simulink model "model"  (R2014a)
(part 5 of 6)

  bus58 : powerlib/Measurements/Load Flow Bus  LConnTagsString=a  ID=bus58  Vbase=110000  Vref=1  Vangle=0  VLF=1  angleLF=0
      settings: AttributesFormatString=|
      | %<ID>
      | %<Vbase>V
      | %<VLF>pu
      | %<angleLF>deg.
      | %<Name>
  bus580 : powerlib/Measurements/Load Flow Bus  LConnTagsString=a  ID=bus580  Vbase=132000  Vref=1  Vangle=0  VLF=1  angleLF=0
      settings: AttributesFormatString=|
      | %<ID>
      | %<Vbase>V
      | %<VLF>pu
      | %<angleLF>deg.
      | %<Name>
  bus581 : powerlib/Measurements/Load Flow Bus  LConnTagsString=a  ID=bus581  Vbase=132000  Vref=1  Vangle=0  VLF=1  angleLF=0
      settings: AttributesFormatString=|
      | %<ID>
      | %<Vbase>V
      | %<VLF>pu
      | %<angleLF>deg.
      | %<Name>
  bus582 : powerlib/Measurements/Load Flow Bus  LConnTagsString=a  ID=bus582  Vbase=132000  Vref=1  Vangle=0  VLF=1  angleLF=0
      settings: AttributesFormatString=|
      | %<ID>
      | %<Vbase>V
      | %<VLF>pu
      | %<angleLF>deg.
      | %<Name>
  bus583 : powerlib/Measurements/Load Flow Bus  LConnTagsString=a  ID=bus583  Vbase=132000  Vref=1  Vangle=0  VLF=1  angleLF=0
      settings: AttributesFormatString=|
      | %<ID>
      | %<Vbase>V
      | %<VLF>pu
      | %<angleLF>deg.
      | %<Name>
  bus584 : powerlib/Measurements/Load Flow Bus  LConnTagsString=a  ID=bus584  Vbase=132000  Vref=1  Vangle=0  VLF=1  angleLF=0
      settings: AttributesFormatString=|
      | %<ID>
      | %<Vbase>V
      | %<VLF>pu
      | %<angleLF>deg.
      | %<Name>
  bus585 : powerlib/Measurements/Load Flow Bus  LConnTagsString=a  ID=bus585  Vbase=132000  Vref=1  Vangle=0  VLF=1  angleLF=0
      settings: AttributesFormatString=|
      | %<ID>
      | %<Vbase>V
      | %<VLF>pu
      | %<angleLF>deg.
      | %<Name>
  bus586 : powerlib/Measurements/Load Flow Bus  LConnTagsString=a  ID=bus586  Vbase=132000  Vref=1  Vangle=0  VLF=1  angleLF=0
      settings: AttributesFormatString=|
      | %<ID>
      | %<Vbase>V
      | %<VLF>pu
      | %<angleLF>deg.
      | %<Name>
  bus587 : powerlib/Measurements/Load Flow Bus  LConnTagsString=a  ID=bus587  Vbase=132000  Vref=1  Vangle=0  VLF=1  angleLF=0
      settings: AttributesFormatString=|
      | %<ID>
      | %<Vbase>V
      | %<VLF>pu
      | %<angleLF>deg.
      | %<Name>
  bus588 : powerlib/Measurements/Load Flow Bus  LConnTagsString=a  ID=bus588  Vbase=132000  Vref=1  Vangle=0  VLF=1  angleLF=0
      settings: AttributesFormatString=|
      | %<ID>
      | %<Vbase>V
      | %<VLF>pu
      | %<angleLF>deg.
      | %<Name>
  bus589 : powerlib/Measurements/Load Flow Bus  LConnTagsString=a  ID=bus589  Vbase=132000  Vref=1  Vangle=0  VLF=1  angleLF=0
      settings: AttributesFormatString=|
      | %<ID>
      | %<Vbase>V
      | %<VLF>pu
      | %<angleLF>deg.
      | %<Name>
  bus59 : powerlib/Measurements/Load Flow Bus  LConnTagsString=a  ID=bus59  Vbase=110000  Vref=1  Vangle=0  VLF=1  angleLF=0
      settings: AttributesFormatString=|
      | %<ID>
      | %<Vbase>V
      | %<VLF>pu
      | %<angleLF>deg.
      | %<Name>
  bus590 : powerlib/Measurements/Load Flow Bus  LConnTagsString=a  ID=bus590  Vbase=132000  Vref=1  Vangle=0  VLF=1  angleLF=0
      settings: AttributesFormatString=|
      | %<ID>
      | %<Vbase>V
      | %<VLF>pu
      | %<angleLF>deg.
      | %<Name>
  bus591 : powerlib/Measurements/Load Flow Bus  LConnTagsString=a  ID=bus591  Vbase=132000  Vref=1  Vangle=0  VLF=1  angleLF=0
      settings: AttributesFormatString=|
      | %<ID>
      | %<Vbase>V
      | %<VLF>pu
      | %<angleLF>deg.
      | %<Name>
  bus592 : powerlib/Measurements/Load Flow Bus  LConnTagsString=a  ID=bus592  Vbase=132000  Vref=1  Vangle=0  VLF=1  angleLF=0
      settings: AttributesFormatString=|
      | %<ID>
      | %<Vbase>V
      | %<VLF>pu
      | %<angleLF>deg.
      | %<Name>
  bus593 : powerlib/Measurements/Load Flow Bus  LConnTagsString=a  ID=bus593  Vbase=132000  Vref=1  Vangle=0  VLF=1  angleLF=0
      settings: AttributesFormatString=|
      | %<ID>
      | %<Vbase>V
      | %<VLF>pu
      | %<angleLF>deg.
      | %<Name>
  bus594 : powerlib/Measurements/Load Flow Bus  LConnTagsString=a  ID=bus594  Vbase=132000  Vref=1  Vangle=0  VLF=1  angleLF=0
      settings: AttributesFormatString=|
      | %<ID>
      | %<Vbase>V
      | %<VLF>pu
      | %<angleLF>deg.
      | %<Name>
  bus595 : powerlib/Measurements/Load Flow Bus  LConnTagsString=a  ID=bus595  Vbase=132000  Vref=1  Vangle=0  VLF=1  angleLF=0
      settings: AttributesFormatString=|
      | %<ID>
      | %<Vbase>V
      | %<VLF>pu
      | %<angleLF>deg.
      | %<Name>
  bus596 : powerlib/Measurements/Load Flow Bus  LConnTagsString=a  ID=bus596  Vbase=132000  Vref=1  Vangle=0  VLF=1  angleLF=0
      settings: AttributesFormatString=|
      | %<ID>
      | %<Vbase>V
      | %<VLF>pu
      | %<angleLF>deg.
      | %<Name>
  bus597 : powerlib/Measurements/Load Flow Bus  LConnTagsString=a  ID=bus597  Vbase=132000  Vref=1  Vangle=0  VLF=1  angleLF=0
      settings: AttributesFormatString=|
      | %<ID>
      | %<Vbase>V
      | %<VLF>pu
      | %<angleLF>deg.
      | %<Name>
  bus598 : powerlib/Measurements/Load Flow Bus  LConnTagsString=a  ID=bus598  Vbase=132000  Vref=1  Vangle=0  VLF=1  angleLF=0
      settings: AttributesFormatString=|
      | %<ID>
      | %<Vbase>V
      | %<VLF>pu
      | %<angleLF>deg.
      | %<Name>
  bus599 : powerlib/Measurements/Load Flow Bus  LConnTagsString=a  ID=bus599  Vbase=132000  Vref=1  Vangle=0  VLF=1  angleLF=0
      settings: AttributesFormatString=|
      | %<ID>
      | %<Vbase>V
      | %<VLF>pu
      | %<angleLF>deg.
      | %<Name>
  bus6 : powerlib/Measurements/Load Flow Bus  LConnTagsString=a  ID=bus6  Vbase=110000  Vref=1  Vangle=0  VLF=1  angleLF=0
      settings: AttributesFormatString=|
      | %<ID>
      | %<Vbase>V
      | %<VLF>pu
      | %<angleLF>deg.
      | %<Name>
  bus60 : powerlib/Measurements/Load Flow Bus  LConnTagsString=a  ID=bus60  Vbase=110000  Vref=1  Vangle=0  VLF=1  angleLF=0
      settings: AttributesFormatString=|
      | %<ID>
      | %<Vbase>V
      | %<VLF>pu
      | %<angleLF>deg.
      | %<Name>
  bus600 : powerlib/Measurements/Load Flow Bus  LConnTagsString=a  ID=bus600  Vbase=132000  Vref=1  Vangle=0  VLF=1  angleLF=0
      settings: AttributesFormatString=|
      | %<ID>
      | %<Vbase>V
      | %<VLF>pu
      | %<angleLF>deg.
      | %<Name>
  bus601 : powerlib/Measurements/Load Flow Bus  LConnTagsString=a  ID=bus601  Vbase=132000  Vref=1  Vangle=0  VLF=1  angleLF=0
      settings: AttributesFormatString=|
      | %<ID>
      | %<Vbase>V
      | %<VLF>pu
      | %<angleLF>deg.
      | %<Name>
  bus602 : powerlib/Measurements/Load Flow Bus  LConnTagsString=a  ID=bus602  Vbase=132000  Vref=1  Vangle=0  VLF=1  angleLF=0
      settings: AttributesFormatString=|
      | %<ID>
      | %<Vbase>V
      | %<VLF>pu
      | %<angleLF>deg.
      | %<Name>
  bus603 : powerlib/Measurements/Load Flow Bus  LConnTagsString=a  ID=bus603  Vbase=132000  Vref=1  Vangle=0  VLF=1  angleLF=0
      settings: AttributesFormatString=|
      | %<ID>
      | %<Vbase>V
      | %<VLF>pu
      | %<angleLF>deg.
      | %<Name>
  bus604 : powerlib/Measurements/Load Flow Bus  LConnTagsString=a  ID=bus604  Vbase=132000  Vref=1  Vangle=0  VLF=1  angleLF=0
      settings: AttributesFormatString=|
      | %<ID>
      | %<Vbase>V
      | %<VLF>pu
      | %<angleLF>deg.
      | %<Name>
  bus605 : powerlib/Measurements/Load Flow Bus  LConnTagsString=a  ID=bus605  Vbase=132000  Vref=1  Vangle=0  VLF=1  angleLF=0
      settings: AttributesFormatString=|
      | %<ID>
      | %<Vbase>V
      | %<VLF>pu
      | %<angleLF>deg.
      | %<Name>
  bus606 : powerlib/Measurements/Load Flow Bus  LConnTagsString=a  ID=bus606  Vbase=132000  Vref=1  Vangle=0  VLF=1  angleLF=0
      settings: AttributesFormatString=|
      | %<ID>
      | %<Vbase>V
      | %<VLF>pu
      | %<angleLF>deg.
      | %<Name>
  bus607 : powerlib/Measurements/Load Flow Bus  LConnTagsString=a  ID=bus607  Vbase=220000  Vref=1  Vangle=0  VLF=1  angleLF=0
      settings: AttributesFormatString=|
      | %<ID>
      | %<Vbase>V
      | %<VLF>pu
      | %<angleLF>deg.
      | %<Name>
  bus608 : powerlib/Measurements/Load Flow Bus  LConnTagsString=a  ID=bus608  Vbase=220000  Vref=1  Vangle=0  VLF=1  angleLF=0
      settings: AttributesFormatString=|
      | %<ID>
      | %<Vbase>V
      | %<VLF>pu
      | %<angleLF>deg.
      | %<Name>
  bus609 : powerlib/Measurements/Load Flow Bus  LConnTagsString=a  ID=bus609  Vbase=220000  Vref=1  Vangle=0  VLF=1  angleLF=0
      settings: AttributesFormatString=|
      | %<ID>
      | %<Vbase>V
      | %<VLF>pu
      | %<angleLF>deg.
      | %<Name>
  bus61 : powerlib/Measurements/Load Flow Bus  LConnTagsString=a  ID=bus61  Vbase=110000  Vref=1  Vangle=0  VLF=1  angleLF=0
      settings: AttributesFormatString=|
      | %<ID>
      | %<Vbase>V
      | %<VLF>pu
      | %<angleLF>deg.
      | %<Name>
  bus610 : powerlib/Measurements/Load Flow Bus  LConnTagsString=a  ID=bus610  Vbase=220000  Vref=1  Vangle=0  VLF=1  angleLF=0
      settings: AttributesFormatString=|
      | %<ID>
      | %<Vbase>V
      | %<VLF>pu
      | %<angleLF>deg.
      | %<Name>
  bus611 : powerlib/Measurements/Load Flow Bus  LConnTagsString=a  ID=bus611  Vbase=220000  Vref=1  Vangle=0  VLF=1  angleLF=0
      settings: AttributesFormatString=|
      | %<ID>
      | %<Vbase>V
      | %<VLF>pu
      | %<angleLF>deg.
      | %<Name>
  bus612 : powerlib/Measurements/Load Flow Bus  LConnTagsString=a  ID=bus612  Vbase=220000  Vref=1  Vangle=0  VLF=1  angleLF=0
      settings: AttributesFormatString=|
      | %<ID>
      | %<Vbase>V
      | %<VLF>pu
      | %<angleLF>deg.
      | %<Name>
  bus613 : powerlib/Measurements/Load Flow Bus  LConnTagsString=a  ID=bus613  Vbase=220000  Vref=1  Vangle=0  VLF=1  angleLF=0
      settings: AttributesFormatString=|
      | %<ID>
      | %<Vbase>V
      | %<VLF>pu
      | %<angleLF>deg.
      | %<Name>
  bus614 : powerlib/Measurements/Load Flow Bus  LConnTagsString=a  ID=bus614  Vbase=220000  Vref=1  Vangle=0  VLF=1  angleLF=0
      settings: AttributesFormatString=|
      | %<ID>
      | %<Vbase>V
      | %<VLF>pu
      | %<angleLF>deg.
      | %<Name>
  bus615 : powerlib/Measurements/Load Flow Bus  LConnTagsString=a  ID=bus615  Vbase=220000  Vref=1  Vangle=0  VLF=1  angleLF=0
      settings: AttributesFormatString=|
      | %<ID>
      | %<Vbase>V
      | %<VLF>pu
      | %<angleLF>deg.
      | %<Name>
  bus616 : powerlib/Measurements/Load Flow Bus  LConnTagsString=a  ID=bus616  Vbase=220000  Vref=1  Vangle=0  VLF=1  angleLF=0
      settings: AttributesFormatString=|
      | %<ID>
      | %<Vbase>V
      | %<VLF>pu
      | %<angleLF>deg.
      | %<Name>
  bus617 : powerlib/Measurements/Load Flow Bus  LConnTagsString=a  ID=bus617  Vbase=220000  Vref=1  Vangle=0  VLF=1  angleLF=0
      settings: AttributesFormatString=|
      | %<ID>
      | %<Vbase>V
      | %<VLF>pu
      | %<angleLF>deg.
      | %<Name>
  bus618 : powerlib/Measurements/Load Flow Bus  LConnTagsString=a  ID=bus618  Vbase=220000  Vref=1  Vangle=0  VLF=1  angleLF=0
      settings: AttributesFormatString=|
      | %<ID>
      | %<Vbase>V
      | %<VLF>pu
      | %<angleLF>deg.
      | %<Name>
  bus619 : powerlib/Measurements/Load Flow Bus  LConnTagsString=a  ID=bus619  Vbase=220000  Vref=1  Vangle=0  VLF=1  angleLF=0
      settings: AttributesFormatString=|
      | %<ID>
      | %<Vbase>V
      | %<VLF>pu
      | %<angleLF>deg.
      | %<Name>
  bus62 : powerlib/Measurements/Load Flow Bus  LConnTagsString=a  ID=bus62  Vbase=110000  Vref=1  Vangle=0  VLF=1  angleLF=0
      settings: AttributesFormatString=|
      | %<ID>
      | %<Vbase>V
      | %<VLF>pu
      | %<angleLF>deg.
      | %<Name>
  bus620 : powerlib/Measurements/Load Flow Bus  LConnTagsString=a  ID=bus620  Vbase=220000  Vref=1  Vangle=0  VLF=1  angleLF=0
      settings: AttributesFormatString=|
      | %<ID>
      | %<Vbase>V
      | %<VLF>pu
      | %<angleLF>deg.
      | %<Name>
  bus621 : powerlib/Measurements/Load Flow Bus  LConnTagsString=a  ID=bus621  Vbase=220000  Vref=1  Vangle=0  VLF=1  angleLF=0
      settings: AttributesFormatString=|
      | %<ID>
      | %<Vbase>V
      | %<VLF>pu
      | %<angleLF>deg.
      | %<Name>
  bus622 : powerlib/Measurements/Load Flow Bus  LConnTagsString=a  ID=bus622  Vbase=220000  Vref=1  Vangle=0  VLF=1  angleLF=0
      settings: AttributesFormatString=|
      | %<ID>
      | %<Vbase>V
      | %<VLF>pu
      | %<angleLF>deg.
      | %<Name>
  bus623 : powerlib/Measurements/Load Flow Bus  LConnTagsString=a  ID=bus623  Vbase=220000  Vref=1  Vangle=0  VLF=1  angleLF=0
      settings: AttributesFormatString=|
      | %<ID>
      | %<Vbase>V
      | %<VLF>pu
      | %<angleLF>deg.
      | %<Name>
  bus624 : powerlib/Measurements/Load Flow Bus  LConnTagsString=a  ID=bus624  Vbase=220000  Vref=1  Vangle=0  VLF=1  angleLF=0
      settings: AttributesFormatString=|
      | %<ID>
      | %<Vbase>V
      | %<VLF>pu
      | %<angleLF>deg.
      | %<Name>
  bus625 : powerlib/Measurements/Load Flow Bus  LConnTagsString=a  ID=bus625  Vbase=220000  Vref=1  Vangle=0  VLF=1  angleLF=0
      settings: AttributesFormatString=|
      | %<ID>
      | %<Vbase>V
      | %<VLF>pu
      | %<angleLF>deg.
      | %<Name>
  bus626 : powerlib/Measurements/Load Flow Bus  LConnTagsString=a  ID=bus626  Vbase=220000  Vref=1  Vangle=0  VLF=1  angleLF=0
      settings: AttributesFormatString=|
      | %<ID>
      | %<Vbase>V
      | %<VLF>pu
      | %<angleLF>deg.
      | %<Name>
  bus627 : powerlib/Measurements/Load Flow Bus  LConnTagsString=a  ID=bus627  Vbase=220000  Vref=1  Vangle=0  VLF=1  angleLF=0
      settings: AttributesFormatString=|
      | %<ID>
      | %<Vbase>V
      | %<VLF>pu
      | %<angleLF>deg.
      | %<Name>
  bus628 : powerlib/Measurements/Load Flow Bus  LConnTagsString=a  ID=bus628  Vbase=220000  Vref=1  Vangle=0  VLF=1  angleLF=0
      settings: AttributesFormatString=|
      | %<ID>
      | %<Vbase>V
      | %<VLF>pu
      | %<angleLF>deg.
      | %<Name>
  bus629 : powerlib/Measurements/Load Flow Bus  LConnTagsString=a  ID=bus629  Vbase=220000  Vref=1  Vangle=0  VLF=1  angleLF=0
      settings: AttributesFormatString=|
      | %<ID>
      | %<Vbase>V
      | %<VLF>pu
      | %<angleLF>deg.
      | %<Name>
  bus63 : powerlib/Measurements/Load Flow Bus  LConnTagsString=a  ID=bus63  Vbase=110000  Vref=1  Vangle=0  VLF=1  angleLF=0
      settings: AttributesFormatString=|
      | %<ID>
      | %<Vbase>V
      | %<VLF>pu
      | %<angleLF>deg.
      | %<Name>
  bus630 : powerlib/Measurements/Load Flow Bus  LConnTagsString=a  ID=bus630  Vbase=220000  Vref=1  Vangle=0  VLF=1  angleLF=0
      settings: AttributesFormatString=|
      | %<ID>
      | %<Vbase>V
      | %<VLF>pu
      | %<angleLF>deg.
      | %<Name>
  bus631 : powerlib/Measurements/Load Flow Bus  LConnTagsString=a  ID=bus631  Vbase=220000  Vref=1  Vangle=0  VLF=1  angleLF=0
      settings: AttributesFormatString=|
      | %<ID>
      | %<Vbase>V
      | %<VLF>pu
      | %<angleLF>deg.
      | %<Name>
  bus632 : powerlib/Measurements/Load Flow Bus  LConnTagsString=a  ID=bus632  Vbase=220000  Vref=1  Vangle=0  VLF=1  angleLF=0
      settings: AttributesFormatString=|
      | %<ID>
      | %<Vbase>V
      | %<VLF>pu
      | %<angleLF>deg.
      | %<Name>
  bus633 : powerlib/Measurements/Load Flow Bus  LConnTagsString=a  ID=bus633  Vbase=220000  Vref=1  Vangle=0  VLF=1  angleLF=0
      settings: AttributesFormatString=|
      | %<ID>
      | %<Vbase>V
      | %<VLF>pu
      | %<angleLF>deg.
      | %<Name>
  bus634 : powerlib/Measurements/Load Flow Bus  LConnTagsString=a  ID=bus634  Vbase=220000  Vref=1  Vangle=0  VLF=1  angleLF=0
      settings: AttributesFormatString=|
      | %<ID>
      | %<Vbase>V
      | %<VLF>pu
      | %<angleLF>deg.
      | %<Name>
  bus635 : powerlib/Measurements/Load Flow Bus  LConnTagsString=a  ID=bus635  Vbase=220000  Vref=1  Vangle=0  VLF=1  angleLF=0
      settings: AttributesFormatString=|
      | %<ID>
      | %<Vbase>V
      | %<VLF>pu
      | %<angleLF>deg.
      | %<Name>
  bus636 : powerlib/Measurements/Load Flow Bus  LConnTagsString=a  ID=bus636  Vbase=220000  Vref=1  Vangle=0  VLF=1  angleLF=0
      settings: AttributesFormatString=|
      | %<ID>
      | %<Vbase>V
      | %<VLF>pu
      | %<angleLF>deg.
      | %<Name>
  bus637 : powerlib/Measurements/Load Flow Bus  LConnTagsString=a  ID=bus637  Vbase=220000  Vref=1  Vangle=0  VLF=1  angleLF=0
      settings: AttributesFormatString=|
      | %<ID>
      | %<Vbase>V
      | %<VLF>pu
      | %<angleLF>deg.
      | %<Name>
  bus638 : powerlib/Measurements/Load Flow Bus  LConnTagsString=a  ID=bus638  Vbase=220000  Vref=1  Vangle=0  VLF=1  angleLF=0
      settings: AttributesFormatString=|
      | %<ID>
      | %<Vbase>V
      | %<VLF>pu
      | %<angleLF>deg.
      | %<Name>
  bus639 : powerlib/Measurements/Load Flow Bus  LConnTagsString=a  ID=bus639  Vbase=220000  Vref=1  Vangle=0  VLF=1  angleLF=0
      settings: AttributesFormatString=|
      | %<ID>
      | %<Vbase>V
      | %<VLF>pu
      | %<angleLF>deg.
      | %<Name>
  bus64 : powerlib/Measurements/Load Flow Bus  LConnTagsString=a  ID=bus64  Vbase=110000  Vref=1  Vangle=0  VLF=1  angleLF=0
      settings: AttributesFormatString=|
      | %<ID>
      | %<Vbase>V
      | %<VLF>pu
      | %<angleLF>deg.
      | %<Name>
  bus640 : powerlib/Measurements/Load Flow Bus  LConnTagsString=a  ID=bus640  Vbase=220000  Vref=1  Vangle=0  VLF=1  angleLF=0
      settings: AttributesFormatString=|
      | %<ID>
      | %<Vbase>V
      | %<VLF>pu
      | %<angleLF>deg.
      | %<Name>
  bus641 : powerlib/Measurements/Load Flow Bus  LConnTagsString=a  ID=bus641  Vbase=220000  Vref=1  Vangle=0  VLF=1  angleLF=0
      settings: AttributesFormatString=|
      | %<ID>
      | %<Vbase>V
      | %<VLF>pu
      | %<angleLF>deg.
      | %<Name>
  bus642 : powerlib/Measurements/Load Flow Bus  LConnTagsString=a  ID=bus642  Vbase=275000  Vref=1  Vangle=0  VLF=1  angleLF=0
      settings: AttributesFormatString=|
      | %<ID>
      | %<Vbase>V
      | %<VLF>pu
      | %<angleLF>deg.
      | %<Name>
  bus643 : powerlib/Measurements/Load Flow Bus  LConnTagsString=a  ID=bus643  Vbase=275000  Vref=1  Vangle=0  VLF=1  angleLF=0
      settings: AttributesFormatString=|
      | %<ID>
      | %<Vbase>V
      | %<VLF>pu
      | %<angleLF>deg.
      | %<Name>
  bus644 : powerlib/Measurements/Load Flow Bus  LConnTagsString=a  ID=bus644  Vbase=275000  Vref=1  Vangle=0  VLF=1  angleLF=0
      settings: AttributesFormatString=|
      | %<ID>
      | %<Vbase>V
      | %<VLF>pu
      | %<angleLF>deg.
      | %<Name>
  bus645 : powerlib/Measurements/Load Flow Bus  LConnTagsString=a  ID=bus645  Vbase=275000  Vref=1  Vangle=0  VLF=1  angleLF=0
      settings: AttributesFormatString=|
      | %<ID>
      | %<Vbase>V
      | %<VLF>pu
      | %<angleLF>deg.
      | %<Name>
  bus646 : powerlib/Measurements/Load Flow Bus  LConnTagsString=a  ID=bus646  Vbase=275000  Vref=1  Vangle=0  VLF=1  angleLF=0
      settings: AttributesFormatString=|
      | %<ID>
      | %<Vbase>V
      | %<VLF>pu
      | %<angleLF>deg.
      | %<Name>
  bus647 : powerlib/Measurements/Load Flow Bus  LConnTagsString=a  ID=bus647  Vbase=275000  Vref=1  Vangle=0  VLF=1  angleLF=0
      settings: AttributesFormatString=|
      | %<ID>
      | %<Vbase>V
      | %<VLF>pu
      | %<angleLF>deg.
      | %<Name>
  bus648 : powerlib/Measurements/Load Flow Bus  LConnTagsString=a  ID=bus648  Vbase=275000  Vref=1  Vangle=0  VLF=1  angleLF=0
      settings: AttributesFormatString=|
      | %<ID>
      | %<Vbase>V
      | %<VLF>pu
      | %<angleLF>deg.
      | %<Name>
  bus649 : powerlib/Measurements/Load Flow Bus  LConnTagsString=a  ID=bus649  Vbase=275000  Vref=1  Vangle=0  VLF=1  angleLF=0
      settings: AttributesFormatString=|
      | %<ID>
      | %<Vbase>V
      | %<VLF>pu
      | %<angleLF>deg.
      | %<Name>
  bus65 : powerlib/Measurements/Load Flow Bus  LConnTagsString=a  ID=bus65  Vbase=110000  Vref=1  Vangle=0  VLF=1  angleLF=0
      settings: AttributesFormatString=|
      | %<ID>
      | %<Vbase>V
      | %<VLF>pu
      | %<angleLF>deg.
      | %<Name>
  bus650 : powerlib/Measurements/Load Flow Bus  LConnTagsString=a  ID=bus650  Vbase=275000  Vref=1  Vangle=0  VLF=1  angleLF=0
      settings: AttributesFormatString=|
      | %<ID>
      | %<Vbase>V
      | %<VLF>pu
      | %<angleLF>deg.
      | %<Name>
  bus651 : powerlib/Measurements/Load Flow Bus  LConnTagsString=a  ID=bus651  Vbase=275000  Vref=1  Vangle=0  VLF=1  angleLF=0
      settings: AttributesFormatString=|
      | %<ID>
      | %<Vbase>V
      | %<VLF>pu
      | %<angleLF>deg.
      | %<Name>
  bus652 : powerlib/Measurements/Load Flow Bus  LConnTagsString=a  ID=bus652  Vbase=275000  Vref=1  Vangle=0  VLF=1  angleLF=0
      settings: AttributesFormatString=|
      | %<ID>
      | %<Vbase>V
      | %<VLF>pu
      | %<angleLF>deg.
      | %<Name>
  bus653 : powerlib/Measurements/Load Flow Bus  LConnTagsString=a  ID=bus653  Vbase=275000  Vref=1  Vangle=0  VLF=1  angleLF=0
      settings: AttributesFormatString=|
      | %<ID>
      | %<Vbase>V
      | %<VLF>pu
      | %<angleLF>deg.
      | %<Name>
  bus654 : powerlib/Measurements/Load Flow Bus  LConnTagsString=a  ID=bus654  Vbase=275000  Vref=1  Vangle=0  VLF=1  angleLF=0
      settings: AttributesFormatString=|
      | %<ID>
      | %<Vbase>V
      | %<VLF>pu
      | %<angleLF>deg.
      | %<Name>
  bus655 : powerlib/Measurements/Load Flow Bus  LConnTagsString=a  ID=bus655  Vbase=275000  Vref=1  Vangle=0  VLF=1  angleLF=0
      settings: AttributesFormatString=|
      | %<ID>
      | %<Vbase>V
      | %<VLF>pu
      | %<angleLF>deg.
      | %<Name>
  bus656 : powerlib/Measurements/Load Flow Bus  LConnTagsString=a  ID=bus656  Vbase=275000  Vref=1  Vangle=0  VLF=1  angleLF=0
      settings: AttributesFormatString=|
      | %<ID>
      | %<Vbase>V
      | %<VLF>pu
      | %<angleLF>deg.
      | %<Name>
  bus657 : powerlib/Measurements/Load Flow Bus  LConnTagsString=a  ID=bus657  Vbase=275000  Vref=1  Vangle=0  VLF=1  angleLF=0
      settings: AttributesFormatString=|
      | %<ID>
      | %<Vbase>V
      | %<VLF>pu
      | %<angleLF>deg.
      | %<Name>
  bus658 : powerlib/Measurements/Load Flow Bus  LConnTagsString=a  ID=bus658  Vbase=275000  Vref=1  Vangle=0  VLF=1  angleLF=0
      settings: AttributesFormatString=|
      | %<ID>
      | %<Vbase>V
      | %<VLF>pu
      | %<angleLF>deg.
      | %<Name>
  bus659 : powerlib/Measurements/Load Flow Bus  LConnTagsString=a  ID=bus659  Vbase=275000  Vref=1  Vangle=0  VLF=1  angleLF=0
      settings: AttributesFormatString=|
      | %<ID>
      | %<Vbase>V
      | %<VLF>pu
      | %<angleLF>deg.
      | %<Name>
  bus66 : powerlib/Measurements/Load Flow Bus  LConnTagsString=a  ID=bus66  Vbase=110000  Vref=1  Vangle=0  VLF=1  angleLF=0
      settings: AttributesFormatString=|
      | %<ID>
      | %<Vbase>V
      | %<VLF>pu
      | %<angleLF>deg.
      | %<Name>
  bus660 : powerlib/Measurements/Load Flow Bus  LConnTagsString=a  ID=bus660  Vbase=275000  Vref=1  Vangle=0  VLF=1  angleLF=0
      settings: AttributesFormatString=|
      | %<ID>
      | %<Vbase>V
      | %<VLF>pu
      | %<angleLF>deg.
      | %<Name>
  bus661 : powerlib/Measurements/Load Flow Bus  LConnTagsString=a  ID=bus661  Vbase=275000  Vref=1  Vangle=0  VLF=1  angleLF=0
      settings: AttributesFormatString=|
      | %<ID>
      | %<Vbase>V
      | %<VLF>pu
      | %<angleLF>deg.
      | %<Name>
  bus662 : powerlib/Measurements/Load Flow Bus  LConnTagsString=a  ID=bus662  Vbase=275000  Vref=1  Vangle=0  VLF=1  angleLF=0
      settings: AttributesFormatString=|
      | %<ID>
      | %<Vbase>V
      | %<VLF>pu
      | %<angleLF>deg.
      | %<Name>
  bus663 : powerlib/Measurements/Load Flow Bus  LConnTagsString=a  ID=bus663  Vbase=275000  Vref=1  Vangle=0  VLF=1  angleLF=0
      settings: AttributesFormatString=|
      | %<ID>
      | %<Vbase>V
      | %<VLF>pu
      | %<angleLF>deg.
      | %<Name>
  bus664 : powerlib/Measurements/Load Flow Bus  LConnTagsString=a  ID=bus664  Vbase=275000  Vref=1  Vangle=0  VLF=1  angleLF=0
      settings: AttributesFormatString=|
      | %<ID>
      | %<Vbase>V
      | %<VLF>pu
      | %<angleLF>deg.
      | %<Name>
  bus665 : powerlib/Measurements/Load Flow Bus  LConnTagsString=a  ID=bus665  Vbase=275000  Vref=1  Vangle=0  VLF=1  angleLF=0
      settings: AttributesFormatString=|
      | %<ID>
      | %<Vbase>V
      | %<VLF>pu
      | %<angleLF>deg.
      | %<Name>
  bus666 : powerlib/Measurements/Load Flow Bus  LConnTagsString=a  ID=bus666  Vbase=330000  Vref=1  Vangle=0  VLF=1  angleLF=0
      settings: AttributesFormatString=|
      | %<ID>
      | %<Vbase>V
      | %<VLF>pu
      | %<angleLF>deg.
      | %<Name>
  bus667 : powerlib/Measurements/Load Flow Bus  LConnTagsString=a  ID=bus667  Vbase=330000  Vref=1  Vangle=0  VLF=1  angleLF=0
      settings: AttributesFormatString=|
      | %<ID>
      | %<Vbase>V
      | %<VLF>pu
      | %<angleLF>deg.
      | %<Name>
  bus668 : powerlib/Measurements/Load Flow Bus  LConnTagsString=a  ID=bus668  Vbase=330000  Vref=1  Vangle=0  VLF=1  angleLF=0
      settings: AttributesFormatString=|
      | %<ID>
      | %<Vbase>V
      | %<VLF>pu
      | %<angleLF>deg.
      | %<Name>
  bus669 : powerlib/Measurements/Load Flow Bus  LConnTagsString=a  ID=bus669  Vbase=330000  Vref=1  Vangle=0  VLF=1  angleLF=0
      settings: AttributesFormatString=|
      | %<ID>
      | %<Vbase>V
      | %<VLF>pu
      | %<angleLF>deg.
      | %<Name>
  bus67 : powerlib/Measurements/Load Flow Bus  LConnTagsString=a  ID=bus67  Vbase=110000  Vref=1  Vangle=0  VLF=1  angleLF=0
      settings: AttributesFormatString=|
      | %<ID>
      | %<Vbase>V
      | %<VLF>pu
      | %<angleLF>deg.
      | %<Name>
  bus670 : powerlib/Measurements/Load Flow Bus  LConnTagsString=a  ID=bus670  Vbase=330000  Vref=1  Vangle=0  VLF=1  angleLF=0
      settings: AttributesFormatString=|
      | %<ID>
      | %<Vbase>V
      | %<VLF>pu
      | %<angleLF>deg.
      | %<Name>
  bus671 : powerlib/Measurements/Load Flow Bus  LConnTagsString=a  ID=bus671  Vbase=330000  Vref=1  Vangle=0  VLF=1  angleLF=0
      settings: AttributesFormatString=|
      | %<ID>
      | %<Vbase>V
      | %<VLF>pu
      | %<angleLF>deg.
      | %<Name>
  bus672 : powerlib/Measurements/Load Flow Bus  LConnTagsString=a  ID=bus672  Vbase=330000  Vref=1  Vangle=0  VLF=1  angleLF=0
      settings: AttributesFormatString=|
      | %<ID>
      | %<Vbase>V
      | %<VLF>pu
      | %<angleLF>deg.
      | %<Name>
  bus673 : powerlib/Measurements/Load Flow Bus  LConnTagsString=a  ID=bus673  Vbase=330000  Vref=1  Vangle=0  VLF=1  angleLF=0
      settings: AttributesFormatString=|
      | %<ID>
      | %<Vbase>V
      | %<VLF>pu
      | %<angleLF>deg.
      | %<Name>
  bus674 : powerlib/Measurements/Load Flow Bus  LConnTagsString=a  ID=bus674  Vbase=330000  Vref=1  Vangle=0  VLF=1  angleLF=0
      settings: AttributesFormatString=|
      | %<ID>
      | %<Vbase>V
      | %<VLF>pu
      | %<angleLF>deg.
      | %<Name>
  bus675 : powerlib/Measurements/Load Flow Bus  LConnTagsString=a  ID=bus675  Vbase=330000  Vref=1  Vangle=0  VLF=1  angleLF=0
      settings: AttributesFormatString=|
      | %<ID>
      | %<Vbase>V
      | %<VLF>pu
      | %<angleLF>deg.
      | %<Name>
  bus676 : powerlib/Measurements/Load Flow Bus  LConnTagsString=a  ID=bus676  Vbase=330000  Vref=1  Vangle=0  VLF=1  angleLF=0
      settings: AttributesFormatString=|
      | %<ID>
      | %<Vbase>V
      | %<VLF>pu
      | %<angleLF>deg.
      | %<Name>
  bus677 : powerlib/Measurements/Load Flow Bus  LConnTagsString=a  ID=bus677  Vbase=330000  Vref=1  Vangle=0  VLF=1  angleLF=0
      settings: AttributesFormatString=|
      | %<ID>
      | %<Vbase>V
      | %<VLF>pu
      | %<angleLF>deg.
      | %<Name>
  bus678 : powerlib/Measurements/Load Flow Bus  LConnTagsString=a  ID=bus678  Vbase=330000  Vref=1  Vangle=0  VLF=1  angleLF=0
      settings: AttributesFormatString=|
      | %<ID>
      | %<Vbase>V
      | %<VLF>pu
      | %<angleLF>deg.
      | %<Name>
  bus679 : powerlib/Measurements/Load Flow Bus  LConnTagsString=a  ID=bus679  Vbase=330000  Vref=1  Vangle=0  VLF=1  angleLF=0
      settings: AttributesFormatString=|
      | %<ID>
      | %<Vbase>V
      | %<VLF>pu
      | %<angleLF>deg.
      | %<Name>
  bus68 : powerlib/Measurements/Load Flow Bus  LConnTagsString=a  ID=bus68  Vbase=132000  Vref=1  Vangle=0  VLF=1  angleLF=0
      settings: AttributesFormatString=|
      | %<ID>
      | %<Vbase>V
      | %<VLF>pu
      | %<angleLF>deg.
      | %<Name>
  bus680 : powerlib/Measurements/Load Flow Bus  LConnTagsString=a  ID=bus680  Vbase=330000  Vref=1  Vangle=0  VLF=1  angleLF=0
      settings: AttributesFormatString=|
      | %<ID>
      | %<Vbase>V
      | %<VLF>pu
      | %<angleLF>deg.
      | %<Name>
  bus681 : powerlib/Measurements/Load Flow Bus  LConnTagsString=a  ID=bus681  Vbase=330000  Vref=1  Vangle=0  VLF=1  angleLF=0
      settings: AttributesFormatString=|
      | %<ID>
      | %<Vbase>V
      | %<VLF>pu
      | %<angleLF>deg.
      | %<Name>
  bus682 : powerlib/Measurements/Load Flow Bus  LConnTagsString=a  ID=bus682  Vbase=330000  Vref=1  Vangle=0  VLF=1  angleLF=0
      settings: AttributesFormatString=|
      | %<ID>
      | %<Vbase>V
      | %<VLF>pu
      | %<angleLF>deg.
      | %<Name>
  bus683 : powerlib/Measurements/Load Flow Bus  LConnTagsString=a  ID=bus683  Vbase=330000  Vref=1  Vangle=0  VLF=1  angleLF=0
      settings: AttributesFormatString=|
      | %<ID>
      | %<Vbase>V
      | %<VLF>pu
      | %<angleLF>deg.
      | %<Name>
  bus684 : powerlib/Measurements/Load Flow Bus  LConnTagsString=a  ID=bus684  Vbase=330000  Vref=1  Vangle=0  VLF=1  angleLF=0
      settings: AttributesFormatString=|
      | %<ID>
      | %<Vbase>V
      | %<VLF>pu
      | %<angleLF>deg.
      | %<Name>
  bus685 : powerlib/Measurements/Load Flow Bus  LConnTagsString=a  ID=bus685  Vbase=330000  Vref=1  Vangle=0  VLF=1  angleLF=0
      settings: AttributesFormatString=|
      | %<ID>
      | %<Vbase>V
      | %<VLF>pu
      | %<angleLF>deg.
      | %<Name>
  bus686 : powerlib/Measurements/Load Flow Bus  LConnTagsString=a  ID=bus686  Vbase=330000  Vref=1  Vangle=0  VLF=1  angleLF=0
      settings: AttributesFormatString=|
      | %<ID>
      | %<Vbase>V
      | %<VLF>pu
      | %<angleLF>deg.
      | %<Name>
  bus687 : powerlib/Measurements/Load Flow Bus  LConnTagsString=a  ID=bus687  Vbase=330000  Vref=1  Vangle=0  VLF=1  angleLF=0
      settings: AttributesFormatString=|
      | %<ID>
      | %<Vbase>V
      | %<VLF>pu
      | %<angleLF>deg.
      | %<Name>
  bus688 : powerlib/Measurements/Load Flow Bus  LConnTagsString=a  ID=bus688  Vbase=330000  Vref=1  Vangle=0  VLF=1  angleLF=0
      settings: AttributesFormatString=|
      | %<ID>
      | %<Vbase>V
      | %<VLF>pu
      | %<angleLF>deg.
      | %<Name>
  bus689 : powerlib/Measurements/Load Flow Bus  LConnTagsString=a  ID=bus689  Vbase=500000  Vref=1  Vangle=0  VLF=1  angleLF=0
      settings: AttributesFormatString=|
      | %<ID>
      | %<Vbase>V
      | %<VLF>pu
      | %<angleLF>deg.
      | %<Name>
  bus69 : powerlib/Measurements/Load Flow Bus  LConnTagsString=a  ID=bus69  Vbase=132000  Vref=1  Vangle=0  VLF=1  angleLF=0
      settings: AttributesFormatString=|
      | %<ID>
      | %<Vbase>V
      | %<VLF>pu
      | %<angleLF>deg.
      | %<Name>
  bus690 : powerlib/Measurements/Load Flow Bus  LConnTagsString=a  ID=bus690  Vbase=500000  Vref=1  Vangle=0  VLF=1  angleLF=0
      settings: AttributesFormatString=|
      | %<ID>
      | %<Vbase>V
      | %<VLF>pu
      | %<angleLF>deg.
      | %<Name>
  bus691 : powerlib/Measurements/Load Flow Bus  LConnTagsString=a  ID=bus691  Vbase=500000  Vref=1  Vangle=0  VLF=1  angleLF=0
      settings: AttributesFormatString=|
      | %<ID>
      | %<Vbase>V
      | %<VLF>pu
      | %<angleLF>deg.
      | %<Name>
  bus692 : powerlib/Measurements/Load Flow Bus  LConnTagsString=a  ID=bus692  Vbase=500000  Vref=1  Vangle=0  VLF=1  angleLF=0
      settings: AttributesFormatString=|
      | %<ID>
      | %<Vbase>V
      | %<VLF>pu
      | %<angleLF>deg.
      | %<Name>
  bus693 : powerlib/Measurements/Load Flow Bus  LConnTagsString=a  ID=bus693  Vbase=500000  Vref=1  Vangle=0  VLF=1  angleLF=0
      settings: AttributesFormatString=|
      | %<ID>
      | %<Vbase>V
      | %<VLF>pu
      | %<angleLF>deg.
      | %<Name>
  bus694 : powerlib/Measurements/Load Flow Bus  LConnTagsString=a  ID=bus694  Vbase=500000  Vref=1  Vangle=0  VLF=1  angleLF=0
      settings: AttributesFormatString=|
      | %<ID>
      | %<Vbase>V
      | %<VLF>pu
      | %<angleLF>deg.
      | %<Name>
  bus7 : powerlib/Measurements/Load Flow Bus  LConnTagsString=a  ID=bus7  Vbase=110000  Vref=1  Vangle=0  VLF=1  angleLF=0
      settings: AttributesFormatString=|
      | %<ID>
      | %<Vbase>V
      | %<VLF>pu
      | %<angleLF>deg.
      | %<Name>
  bus70 : powerlib/Measurements/Load Flow Bus  LConnTagsString=a  ID=bus70  Vbase=132000  Vref=1  Vangle=0  VLF=1  angleLF=0
      settings: AttributesFormatString=|
      | %<ID>
      | %<Vbase>V
      | %<VLF>pu
      | %<angleLF>deg.
      | %<Name>
  bus71 : powerlib/Measurements/Load Flow Bus  LConnTagsString=a  ID=bus71  Vbase=132000  Vref=1  Vangle=0  VLF=1  angleLF=0
      settings: AttributesFormatString=|
      | %<ID>
      | %<Vbase>V
      | %<VLF>pu
      | %<angleLF>deg.
      | %<Name>
  bus72 : powerlib/Measurements/Load Flow Bus  LConnTagsString=a  ID=bus72  Vbase=132000  Vref=1  Vangle=0  VLF=1  angleLF=0
      settings: AttributesFormatString=|
      | %<ID>
      | %<Vbase>V
      | %<VLF>pu
      | %<angleLF>deg.
      | %<Name>
  bus73 : powerlib/Measurements/Load Flow Bus  LConnTagsString=a  ID=bus73  Vbase=132000  Vref=1  Vangle=0  VLF=1  angleLF=0
      settings: AttributesFormatString=|
      | %<ID>
      | %<Vbase>V
      | %<VLF>pu
      | %<angleLF>deg.
      | %<Name>
  bus74 : powerlib/Measurements/Load Flow Bus  LConnTagsString=a  ID=bus74  Vbase=132000  Vref=1  Vangle=0  VLF=1  angleLF=0
      settings: AttributesFormatString=|
      | %<ID>
      | %<Vbase>V
      | %<VLF>pu
      | %<angleLF>deg.
      | %<Name>
  bus75 : powerlib/Measurements/Load Flow Bus  LConnTagsString=a  ID=bus75  Vbase=132000  Vref=1  Vangle=0  VLF=1  angleLF=0
      settings: AttributesFormatString=|
      | %<ID>
      | %<Vbase>V
      | %<VLF>pu
      | %<angleLF>deg.
      | %<Name>
  bus76 : powerlib/Measurements/Load Flow Bus  LConnTagsString=a  ID=bus76  Vbase=132000  Vref=1  Vangle=0  VLF=1  angleLF=0
      settings: AttributesFormatString=|
      | %<ID>
      | %<Vbase>V
      | %<VLF>pu
      | %<angleLF>deg.
      | %<Name>
  bus77 : powerlib/Measurements/Load Flow Bus  LConnTagsString=a  ID=bus77  Vbase=132000  Vref=1  Vangle=0  VLF=1  angleLF=0
      settings: AttributesFormatString=|
      | %<ID>
      | %<Vbase>V
      | %<VLF>pu
      | %<angleLF>deg.
      | %<Name>
  bus78 : powerlib/Measurements/Load Flow Bus  LConnTagsString=a  ID=bus78  Vbase=132000  Vref=1  Vangle=0  VLF=1  angleLF=0
      settings: AttributesFormatString=|
      | %<ID>
      | %<Vbase>V
      | %<VLF>pu
      | %<angleLF>deg.
      | %<Name>
  bus79 : powerlib/Measurements/Load Flow Bus  LConnTagsString=a  ID=bus79  Vbase=132000  Vref=1  Vangle=0  VLF=1  angleLF=0
      settings: AttributesFormatString=|
      | %<ID>
      | %<Vbase>V
      | %<VLF>pu
      | %<angleLF>deg.
      | %<Name>
  bus8 : powerlib/Measurements/Load Flow Bus  LConnTagsString=a  ID=bus8  Vbase=110000  Vref=1  Vangle=0  VLF=1  angleLF=0
      settings: AttributesFormatString=|
      | %<ID>
      | %<Vbase>V
      | %<VLF>pu
      | %<angleLF>deg.
      | %<Name>
  bus80 : powerlib/Measurements/Load Flow Bus  LConnTagsString=a  ID=bus80  Vbase=132000  Vref=1  Vangle=0  VLF=1  angleLF=0
      settings: AttributesFormatString=|
      | %<ID>
      | %<Vbase>V
      | %<VLF>pu
      | %<angleLF>deg.
      | %<Name>
  bus81 : powerlib/Measurements/Load Flow Bus  LConnTagsString=a  ID=bus81  Vbase=132000  Vref=1  Vangle=0  VLF=1  angleLF=0
      settings: AttributesFormatString=|
      | %<ID>
      | %<Vbase>V
      | %<VLF>pu
      | %<angleLF>deg.
      | %<Name>
  bus82 : powerlib/Measurements/Load Flow Bus  LConnTagsString=a  ID=bus82  Vbase=132000  Vref=1  Vangle=0  VLF=1  angleLF=0
      settings: AttributesFormatString=|
      | %<ID>
      | %<Vbase>V
      | %<VLF>pu
      | %<angleLF>deg.
      | %<Name>
  bus83 : powerlib/Measurements/Load Flow Bus  LConnTagsString=a  ID=bus83  Vbase=132000  Vref=1  Vangle=0  VLF=1  angleLF=0
      settings: AttributesFormatString=|
      | %<ID>
      | %<Vbase>V
      | %<VLF>pu
      | %<angleLF>deg.
      | %<Name>
  bus84 : powerlib/Measurements/Load Flow Bus  LConnTagsString=a  ID=bus84  Vbase=132000  Vref=1  Vangle=0  VLF=1  angleLF=0
      settings: AttributesFormatString=|
      | %<ID>
      | %<Vbase>V
      | %<VLF>pu
      | %<angleLF>deg.
      | %<Name>
  bus85 : powerlib/Measurements/Load Flow Bus  LConnTagsString=a  ID=bus85  Vbase=132000  Vref=1  Vangle=0  VLF=1  angleLF=0
      settings: AttributesFormatString=|
      | %<ID>
      | %<Vbase>V
      | %<VLF>pu
      | %<angleLF>deg.
      | %<Name>
  bus86 : powerlib/Measurements/Load Flow Bus  LConnTagsString=a  ID=bus86  Vbase=132000  Vref=1  Vangle=0  VLF=1  angleLF=0
      settings: AttributesFormatString=|
      | %<ID>
      | %<Vbase>V
      | %<VLF>pu
      | %<angleLF>deg.
      | %<Name>
  bus87 : powerlib/Measurements/Load Flow Bus  LConnTagsString=a  ID=bus87  Vbase=132000  Vref=1  Vangle=0  VLF=1  angleLF=0
      settings: AttributesFormatString=|
      | %<ID>
      | %<Vbase>V
      | %<VLF>pu
      | %<angleLF>deg.
      | %<Name>
  bus88 : powerlib/Measurements/Load Flow Bus  LConnTagsString=a  ID=bus88  Vbase=132000  Vref=1  Vangle=0  VLF=1  angleLF=0
      settings: AttributesFormatString=|
      | %<ID>
      | %<Vbase>V
      | %<VLF>pu
      | %<angleLF>deg.
      | %<Name>
  bus89 : powerlib/Measurements/Load Flow Bus  LConnTagsString=a  ID=bus89  Vbase=132000  Vref=1  Vangle=0  VLF=1  angleLF=0
      settings: AttributesFormatString=|
      | %<ID>
      | %<Vbase>V
      | %<VLF>pu
      | %<angleLF>deg.
      | %<Name>
  bus9 : powerlib/Measurements/Load Flow Bus  LConnTagsString=a  ID=bus9  Vbase=110000  Vref=1  Vangle=0  VLF=1  angleLF=0
      settings: AttributesFormatString=|
      | %<ID>
      | %<Vbase>V
      | %<VLF>pu
      | %<angleLF>deg.
      | %<Name>
  bus90 : powerlib/Measurements/Load Flow Bus  LConnTagsString=a  ID=bus90  Vbase=132000  Vref=1  Vangle=0  VLF=1  angleLF=0
      settings: AttributesFormatString=|
      | %<ID>
      | %<Vbase>V
      | %<VLF>pu
      | %<angleLF>deg.
      | %<Name>
  bus91 : powerlib/Measurements/Load Flow Bus  LConnTagsString=a  ID=bus91  Vbase=132000  Vref=1  Vangle=0  VLF=1  angleLF=0
      settings: AttributesFormatString=|
      | %<ID>
      | %<Vbase>V
      | %<VLF>pu
      | %<angleLF>deg.
      | %<Name>
  bus92 : powerlib/Measurements/Load Flow Bus  LConnTagsString=a  ID=bus92  Vbase=132000  Vref=1  Vangle=0  VLF=1  angleLF=0
      settings: AttributesFormatString=|
      | %<ID>
      | %<Vbase>V
      | %<VLF>pu
      | %<angleLF>deg.
      | %<Name>
  bus93 : powerlib/Measurements/Load Flow Bus  LConnTagsString=a  ID=bus93  Vbase=132000  Vref=1  Vangle=0  VLF=1  angleLF=0
      settings: AttributesFormatString=|
      | %<ID>
      | %<Vbase>V
      | %<VLF>pu
      | %<angleLF>deg.
      | %<Name>
  bus94 : powerlib/Measurements/Load Flow Bus  LConnTagsString=a  ID=bus94  Vbase=132000  Vref=1  Vangle=0  VLF=1  angleLF=0
      settings: AttributesFormatString=|
      | %<ID>
      | %<Vbase>V
      | %<VLF>pu
      | %<angleLF>deg.
      | %<Name>
  bus95 : powerlib/Measurements/Load Flow Bus  LConnTagsString=a  ID=bus95  Vbase=132000  Vref=1  Vangle=0  VLF=1  angleLF=0
      settings: AttributesFormatString=|
      | %<ID>
      | %<Vbase>V
      | %<VLF>pu
      | %<angleLF>deg.
      | %<Name>
  bus96 : powerlib/Measurements/Load Flow Bus  LConnTagsString=a  ID=bus96  Vbase=132000  Vref=1  Vangle=0  VLF=1  angleLF=0
      settings: AttributesFormatString=|
      | %<ID>
      | %<Vbase>V
      | %<VLF>pu
      | %<angleLF>deg.
      | %<Name>
  bus97 : powerlib/Measurements/Load Flow Bus  LConnTagsString=a  ID=bus97  Vbase=132000  Vref=1  Vangle=0  VLF=1  angleLF=0
      settings: AttributesFormatString=|
      | %<ID>
      | %<Vbase>V
      | %<VLF>pu
      | %<angleLF>deg.
      | %<Name>
  bus98 : powerlib/Measurements/Load Flow Bus  LConnTagsString=a  ID=bus98  Vbase=132000  Vref=1  Vangle=0  VLF=1  angleLF=0
      settings: AttributesFormatString=|
      | %<ID>
      | %<Vbase>V
      | %<VLF>pu
      | %<angleLF>deg.
      | %<Name>
  bus99 : powerlib/Measurements/Load Flow Bus  LConnTagsString=a  ID=bus99  Vbase=132000  Vref=1  Vangle=0  VLF=1  angleLF=0
      settings: AttributesFormatString=|
      | %<ID>
      | %<Vbase>V
      | %<VLF>pu
      | %<angleLF>deg.
      | %<Name>
  powergui : powerlib/powergui  Priority=1  SimulationMode=Continuous  SolverType=Tustin  SampleTime=50e-6  frequency=60  SPID=off  DisableSnubberDevices=off  DisableRonSwitches=off  DisableVfSwitches=off  SwTol=0  Interpol=off  DisplayEquations=off  Ts=0  methode=off  frequencyindice=60  Pbase=100e6  ErrMax=1e-4  Iterations=50  UnitsV=kV  UnitsW=MW  FunctionMessages=off  echomessages=off  HookPort=off  EnableUseOfTLC=off  x0status=blocks  RestoreLinks=warning  ResistiveCurrentMeasurement=off  Frange=[0:2:500]  Ylog=off  Xlog=on  ShowGrid=off  save=off  variable=ZData  structure=0  ZoomFFT=off  StartTime=0.0  cycles=1  DisplayStyle=1  fundamental=60  FreqAxis=off  MaxFrequency=1000  frequencyindicesteady=1  RmsSteady=1  display=off
  connections:
  T_305092097__/LConn1 -- _CN_305092097_110000_CN_305092094_110000/LConn1
  T_305092097__/LConn2 -- _CN_305092097_110000_CN_305092094_110000/LConn2
  _CN_305092097_110000_CN_305092094_110000/LConn3 -- T_305092097__/LConn3 -- bus1/LConn1
  T_305092094__/LConn1 -- _CN_305092097_110000_CN_305092094_110000/RConn1
  T_305092094__/LConn2 -- _CN_305092097_110000_CN_305092094_110000/RConn2
  _CN_305092097_110000_CN_305092094_110000/RConn3 -- T_305092094__/LConn3 -- bus2/LConn1
  _CN_88187651_110000_CN_61649117_110000/LConn1 -- T_88187651__Hadspen_Substation/RConn1 -- _CN_88187651_110000_CN_174441055_110000/LConn1 -- L_88187651/LConn1
  _CN_88187651_110000_CN_61649117_110000/LConn2 -- T_88187651__Hadspen_Substation/RConn2 -- _CN_88187651_110000_CN_174441055_110000/LConn2 -- L_88187651/LConn2
  _CN_88187651_110000_CN_61649117_110000/LConn3 -- T_88187651__Hadspen_Substation/RConn3 -- _CN_88187651_110000_CN_174441055_110000/LConn3 -- L_88187651/LConn3 -- bus3/LConn1
  G_61649117_Trevallyn_Power_Station/RConn1 -- _CN_88187651_110000_CN_61649117_110000/RConn1
  G_61649117_Trevallyn_Power_Station/RConn2 -- _CN_88187651_110000_CN_61649117_110000/RConn2
  _CN_88187651_110000_CN_61649117_110000/RConn3 -- G_61649117_Trevallyn_Power_Station/RConn3 -- bus4/LConn1
  _CN_88187651_110000_CN_174441055_110000/RConn1 -- T_174441055__/RConn1 -- L_174441055/LConn1
  _CN_88187651_110000_CN_174441055_110000/RConn2 -- T_174441055__/RConn2 -- L_174441055/LConn2
  _CN_88187651_110000_CN_174441055_110000/RConn3 -- T_174441055__/RConn3 -- L_174441055/LConn3 -- bus5/LConn1
  _CN_303420374_110000_CN_46146107_110000/LConn1 -- T_303420374__Richlands_Substation/LConn1 -- _CN_303420374_110000_CN_19388439_110000/LConn1 -- _CN_303420374_110000_CN_303417152_110000/LConn1
  _CN_303420374_110000_CN_46146107_110000/LConn2 -- T_303420374__Richlands_Substation/LConn2 -- _CN_303420374_110000_CN_19388439_110000/LConn2 -- _CN_303420374_110000_CN_303417152_110000/LConn2
  _CN_303420374_110000_CN_46146107_110000/LConn3 -- T_303420374__Richlands_Substation/LConn3 -- _CN_303420374_110000_CN_19388439_110000/LConn3 -- _CN_303420374_110000_CN_303417152_110000/LConn3 -- bus6/LConn1
  _CN_303420374_110000_CN_46146107_110000/RConn1 -- T_46146107__Algester_Substation/LConn1 -- _CN_26161587_110000_CN_46146107_110000/LConn1
  _CN_303420374_110000_CN_46146107_110000/RConn2 -- T_46146107__Algester_Substation/LConn2 -- _CN_26161587_110000_CN_46146107_110000/LConn2
  _CN_303420374_110000_CN_46146107_110000/RConn3 -- T_46146107__Algester_Substation/LConn3 -- _CN_26161587_110000_CN_46146107_110000/LConn3 -- bus7/LConn1
  _CN_303420374_110000_CN_19388439_110000/RConn1 -- T_19388439__West_Darra_Substation/LConn1 -- _CN_19388439_110000_CN_173223683_110000/LConn1 -- _CN_19388439_110000_CN_19386719_110000/LConn1 -- _CN_19388439_110000_CN_46305863_110000/LConn1
  _CN_303420374_110000_CN_19388439_110000/RConn2 -- T_19388439__West_Darra_Substation/LConn2 -- _CN_19388439_110000_CN_173223683_110000/LConn2 -- _CN_19388439_110000_CN_19386719_110000/LConn2 -- _CN_19388439_110000_CN_46305863_110000/LConn2
  _CN_303420374_110000_CN_19388439_110000/RConn3 -- T_19388439__West_Darra_Substation/LConn3 -- _CN_19388439_110000_CN_173223683_110000/LConn3 -- _CN_19388439_110000_CN_19386719_110000/LConn3 -- bus8/LConn1 -- _CN_19388439_110000_CN_46305863_110000/LConn3
  T_303417152__Sumner_Substation/LConn1 -- _CN_303420374_110000_CN_303417152_110000/RConn1
  T_303417152__Sumner_Substation/LConn2 -- _CN_303420374_110000_CN_303417152_110000/RConn2
  _CN_303420374_110000_CN_303417152_110000/RConn3 -- T_303417152__Sumner_Substation/LConn3 -- bus9/LConn1
  T_162321863__/LConn1 -- _CN_162321863_110000_CN_19380255_110000/LConn1
  T_162321863__/LConn2 -- _CN_162321863_110000_CN_19380255_110000/LConn2
  _CN_162321863_110000_CN_19380255_110000/LConn3 -- T_162321863__/LConn3 -- bus10/LConn1
  _CN_162321863_110000_CN_19380255_110000/RConn1 -- G_19380255_Swanbank_Power_Station/RConn1 -- _CN_173223683_110000_CN_19380255_110000/LConn1 -- _CN_170832455_275000_CN_19380255_110000/LConn1
  _CN_162321863_110000_CN_19380255_110000/RConn2 -- G_19380255_Swanbank_Power_Station/RConn2 -- _CN_173223683_110000_CN_19380255_110000/LConn2 -- _CN_170832455_275000_CN_19380255_110000/LConn2
  _CN_162321863_110000_CN_19380255_110000/RConn3 -- G_19380255_Swanbank_Power_Station/RConn3 -- _CN_173223683_110000_CN_19380255_110000/LConn3 -- _CN_170832455_275000_CN_19380255_110000/LConn3 -- bus11/LConn1
  T_372546567__/LConn1 -- _CN_372546567_110000_CN_23171307_110000/LConn1
  T_372546567__/LConn2 -- _CN_372546567_110000_CN_23171307_110000/LConn2
  _CN_372546567_110000_CN_23171307_110000/LConn3 -- T_372546567__/LConn3 -- bus12/LConn1
  T_23171307__/LConn1 -- _CN_372546567_110000_CN_23171307_110000/RConn1
  T_23171307__/LConn2 -- _CN_372546567_110000_CN_23171307_110000/RConn2
  _CN_372546567_110000_CN_23171307_110000/RConn3 -- T_23171307__/LConn3 -- bus13/LConn1
  T_233929226__/LConn1 -- _CN_233929226_110000_CN_435794582_110000/LConn1
  T_233929226__/LConn2 -- _CN_233929226_110000_CN_435794582_110000/LConn2
  _CN_233929226_110000_CN_435794582_110000/LConn3 -- T_233929226__/LConn3 -- bus14/LConn1
  _CN_233929226_110000_CN_435794582_110000/RConn1 -- T_435794582__Tungatinah_Switchyard/LConn1 -- _CN_435794582_110000_CN_176275951_110000/LConn1
  _CN_233929226_110000_CN_435794582_110000/RConn2 -- T_435794582__Tungatinah_Switchyard/LConn2 -- _CN_435794582_110000_CN_176275951_110000/LConn2
  _CN_233929226_110000_CN_435794582_110000/RConn3 -- T_435794582__Tungatinah_Switchyard/LConn3 -- _CN_435794582_110000_CN_176275951_110000/LConn3 -- bus15/LConn1
  _CN_23298443_110000_CN_23239876_110000/LConn1 -- T_23298443__/RConn1 -- _CN_23298443_110000_CN_175926350_110000/LConn1 -- _CN_23298443_110000_CN_233927398_110000/LConn1 -- _CN_23298443_110000_CN_233927458_110000/LConn1 -- L_23298443/LConn1
  _CN_23298443_110000_CN_23239876_110000/LConn2 -- T_23298443__/RConn2 -- _CN_23298443_110000_CN_175926350_110000/LConn2 -- _CN_23298443_110000_CN_233927398_110000/LConn2 -- _CN_23298443_110000_CN_233927458_110000/LConn2 -- L_23298443/LConn2
  _CN_23298443_110000_CN_23239876_110000/LConn3 -- T_23298443__/RConn3 -- _CN_23298443_110000_CN_175926350_110000/LConn3 -- _CN_23298443_110000_CN_233927398_110000/LConn3 -- _CN_23298443_110000_CN_233927458_110000/LConn3 -- L_23298443/LConn3 -- bus16/LConn1
  T_23239876__/LConn1 -- _CN_23298443_110000_CN_23239876_110000/RConn1
  T_23239876__/LConn2 -- _CN_23298443_110000_CN_23239876_110000/RConn2
  _CN_23298443_110000_CN_23239876_110000/RConn3 -- T_23239876__/LConn3 -- bus17/LConn1
  _CN_23298443_110000_CN_175926350_110000/RConn1 -- T_175926350__/LConn1 -- _CN_175926345_110000_CN_175926350_110000/LConn1
  _CN_23298443_110000_CN_175926350_110000/RConn2 -- T_175926350__/LConn2 -- _CN_175926345_110000_CN_175926350_110000/LConn2
  _CN_23298443_110000_CN_175926350_110000/RConn3 -- T_175926350__/LConn3 -- _CN_175926345_110000_CN_175926350_110000/LConn3 -- bus18/LConn1
  T_233927398__/LConn1 -- _CN_23298443_110000_CN_233927398_110000/RConn1
  T_233927398__/LConn2 -- _CN_23298443_110000_CN_233927398_110000/RConn2
  _CN_23298443_110000_CN_233927398_110000/RConn3 -- T_233927398__/LConn3 -- bus19/LConn1
  T_233927458__/LConn1 -- _CN_23298443_110000_CN_233927458_110000/RConn1
  T_233927458__/LConn2 -- _CN_23298443_110000_CN_233927458_110000/RConn2
  _CN_23298443_110000_CN_233927458_110000/RConn3 -- T_233927458__/LConn3 -- bus20/LConn1
  T_374644110__/LConn1 -- _CN_374644110_110000_CN_46056595_110000/LConn1
  T_374644110__/LConn2 -- _CN_374644110_110000_CN_46056595_110000/LConn2
  _CN_374644110_110000_CN_46056595_110000/LConn3 -- T_374644110__/LConn3 -- bus21/LConn1
  T_46056595__/LConn1 -- _CN_374644110_110000_CN_46056595_110000/RConn1
  T_46056595__/LConn2 -- _CN_374644110_110000_CN_46056595_110000/RConn2
  _CN_374644110_110000_CN_46056595_110000/RConn3 -- T_46056595__/LConn3 -- bus22/LConn1
  _CN_19384720_110000_CN_171582113_110000/LConn1 -- T_19384720__South_Pine_Substation/RConn1 -- L_19384720/LConn1
  _CN_19384720_110000_CN_171582113_110000/LConn2 -- T_19384720__South_Pine_Substation/RConn2 -- L_19384720/LConn2
  _CN_19384720_110000_CN_171582113_110000/LConn3 -- T_19384720__South_Pine_Substation/RConn3 -- L_19384720/LConn3 -- bus23/LConn1
  T_171582113__/LConn1 -- _CN_19384720_110000_CN_171582113_110000/RConn1
  T_171582113__/LConn2 -- _CN_19384720_110000_CN_171582113_110000/RConn2
  _CN_19384720_110000_CN_171582113_110000/RConn3 -- T_171582113__/LConn3 -- bus24/LConn1
  _CN_308160583_110000_CN_308160585_110000/LConn1 -- T_308160583__Gatton_North_Substation/LConn1 -- _CN_308160583_110000_CN_66035178_110000/LConn1 -- _CN_308160583_110000_CN_173223683_110000/LConn1
  _CN_308160583_110000_CN_308160585_110000/LConn2 -- T_308160583__Gatton_North_Substation/LConn2 -- _CN_308160583_110000_CN_66035178_110000/LConn2 -- _CN_308160583_110000_CN_173223683_110000/LConn2
  _CN_308160583_110000_CN_308160585_110000/LConn3 -- T_308160583__Gatton_North_Substation/LConn3 -- _CN_308160583_110000_CN_66035178_110000/LConn3 -- _CN_308160583_110000_CN_173223683_110000/LConn3 -- bus25/LConn1
  _CN_308160583_110000_CN_308160585_110000/RConn1 -- T_308160585__Postmans_Ridge_Substation/LConn1 -- _CN_172878761_110000_CN_308160585_110000/LConn1
  _CN_308160583_110000_CN_308160585_110000/RConn2 -- T_308160585__Postmans_Ridge_Substation/LConn2 -- _CN_172878761_110000_CN_308160585_110000/LConn2
  _CN_308160583_110000_CN_308160585_110000/RConn3 -- T_308160585__Postmans_Ridge_Substation/LConn3 -- _CN_172878761_110000_CN_308160585_110000/LConn3 -- bus26/LConn1
  T_66035178__Lockrose_Substation/LConn1 -- _CN_308160583_110000_CN_66035178_110000/RConn1
  T_66035178__Lockrose_Substation/LConn2 -- _CN_308160583_110000_CN_66035178_110000/RConn2
  _CN_308160583_110000_CN_66035178_110000/RConn3 -- T_66035178__Lockrose_Substation/LConn3 -- bus27/LConn1
  _CN_308160583_110000_CN_173223683_110000/RConn1 -- T_173223683__Abermain_Substation/RConn1 -- _CN_19388439_110000_CN_173223683_110000/RConn1 -- _CN_173223683_110000_CN_19380255_110000/RConn1 -- L_173223683/LConn1
  _CN_308160583_110000_CN_173223683_110000/RConn2 -- T_173223683__Abermain_Substation/RConn2 -- _CN_19388439_110000_CN_173223683_110000/RConn2 -- _CN_173223683_110000_CN_19380255_110000/RConn2 -- L_173223683/LConn2
  _CN_308160583_110000_CN_173223683_110000/RConn3 -- T_173223683__Abermain_Substation/RConn3 -- _CN_19388439_110000_CN_173223683_110000/RConn3 -- _CN_173223683_110000_CN_19380255_110000/RConn3 -- L_173223683/LConn3 -- bus28/LConn1
  _CN_19388439_110000_CN_46305863_110000/RConn1 -- T_46305863__Goodna_Substation/LConn1 -- _CN_26204314_110000_CN_46305863_110000/LConn1
  _CN_19388439_110000_CN_46305863_110000/RConn2 -- T_46305863__Goodna_Substation/LConn2 -- _CN_26204314_110000_CN_46305863_110000/LConn2
  _CN_19388439_110000_CN_46305863_110000/RConn3 -- T_46305863__Goodna_Substation/LConn3 -- _CN_26204314_110000_CN_46305863_110000/LConn3 -- bus29/LConn1
  T_19386719__/LConn1 -- _CN_19388439_110000_CN_19386719_110000/RConn1
  T_19386719__/LConn2 -- _CN_19388439_110000_CN_19386719_110000/RConn2
  _CN_19388439_110000_CN_19386719_110000/RConn3 -- T_19386719__/LConn3 -- bus30/LConn1
  T_26204314__Redbank_Plains_Substation/LConn1 -- _CN_26204314_110000_CN_46305863_110000/RConn1
  T_26204314__Redbank_Plains_Substation/LConn2 -- _CN_26204314_110000_CN_46305863_110000/RConn2
  _CN_26204314_110000_CN_46305863_110000/RConn3 -- T_26204314__Redbank_Plains_Substation/LConn3 -- bus31/LConn1
  _CN_26230300_110000_CN_26161587_110000/LConn1 -- T_26230300__Belmont_Substation/RConn1 -- _CN_26230300_110000_CN_44418650_110000/LConn1 -- L_26230300/LConn1
  _CN_26230300_110000_CN_26161587_110000/LConn2 -- T_26230300__Belmont_Substation/RConn2 -- _CN_26230300_110000_CN_44418650_110000/LConn2 -- L_26230300/LConn2
  _CN_26230300_110000_CN_26161587_110000/LConn3 -- T_26230300__Belmont_Substation/RConn3 -- _CN_26230300_110000_CN_44418650_110000/LConn3 -- L_26230300/LConn3 -- bus32/LConn1
  _CN_26230300_110000_CN_26161587_110000/RConn1 -- T_26161587__Runcorn_Substation/LConn1 -- _CN_26161587_110000_CN_46146107_110000/RConn1
  _CN_26230300_110000_CN_26161587_110000/RConn2 -- T_26161587__Runcorn_Substation/LConn2 -- _CN_26161587_110000_CN_46146107_110000/RConn2
  _CN_26230300_110000_CN_26161587_110000/RConn3 -- T_26161587__Runcorn_Substation/LConn3 -- _CN_26161587_110000_CN_46146107_110000/RConn3 -- bus33/LConn1
  _CN_26230300_110000_CN_44418650_110000/RConn1 -- T_44418650__/RConn1 -- L_44418650/LConn1
  _CN_26230300_110000_CN_44418650_110000/RConn2 -- T_44418650__/RConn2 -- L_44418650/LConn2
  _CN_26230300_110000_CN_44418650_110000/RConn3 -- T_44418650__/RConn3 -- L_44418650/LConn3 -- bus34/LConn1
  T_234083162__/LConn1 -- Farrell___Waratah_CN_234083162_110000_CN_234083164_110000/LConn1
  T_234083162__/LConn2 -- Farrell___Waratah_CN_234083162_110000_CN_234083164_110000/LConn2
  Farrell___Waratah_CN_234083162_110000_CN_234083164_110000/LConn3 -- T_234083162__/LConn3 -- bus35/LConn1
  Farrell___Waratah_CN_234083162_110000_CN_234083164_110000/RConn1 -- T_234083164__/LConn1 -- Burnie___Waratah_CN_234083164_110000_CN_234083565_110000/LConn1
  Farrell___Waratah_CN_234083162_110000_CN_234083164_110000/RConn2 -- T_234083164__/LConn2 -- Burnie___Waratah_CN_234083164_110000_CN_234083565_110000/LConn2
  Farrell___Waratah_CN_234083162_110000_CN_234083164_110000/RConn3 -- T_234083164__/LConn3 -- Burnie___Waratah_CN_234083164_110000_CN_234083565_110000/LConn3 -- bus36/LConn1
  T_171575462__/LConn1 -- _CN_171575462_110000_CN_171575468_110000/LConn1
  T_171575462__/LConn2 -- _CN_171575462_110000_CN_171575468_110000/LConn2
  _CN_171575462_110000_CN_171575468_110000/LConn3 -- T_171575462__/LConn3 -- bus37/LConn1
  _CN_171575462_110000_CN_171575468_110000/RConn1 -- T_171575468__/LConn1 -- _CN_171575468_110000_CN_172878761_110000/LConn1
  _CN_171575462_110000_CN_171575468_110000/RConn2 -- T_171575468__/LConn2 -- _CN_171575468_110000_CN_172878761_110000/LConn2
  _CN_171575462_110000_CN_171575468_110000/RConn3 -- T_171575468__/LConn3 -- _CN_171575468_110000_CN_172878761_110000/LConn3 -- bus38/LConn1
  _CN_88191017_110000_CN_174431697_110000/LConn1 -- T_88191017__/RConn1 -- _CN_88191017_110000_CN_175174348_110000/LConn1 -- _CN_88191017_110000_CN_167791635_110000/LConn1 -- L_88191017/LConn1
  _CN_88191017_110000_CN_174431697_110000/LConn2 -- T_88191017__/RConn2 -- _CN_88191017_110000_CN_175174348_110000/LConn2 -- _CN_88191017_110000_CN_167791635_110000/LConn2 -- L_88191017/LConn2
  _CN_88191017_110000_CN_174431697_110000/LConn3 -- T_88191017__/RConn3 -- _CN_88191017_110000_CN_175174348_110000/LConn3 -- _CN_88191017_110000_CN_167791635_110000/LConn3 -- L_88191017/LConn3 -- bus39/LConn1
  T_174431697__Devonport_Substation/LConn1 -- _CN_88191017_110000_CN_174431697_110000/RConn1
  T_174431697__Devonport_Substation/LConn2 -- _CN_88191017_110000_CN_174431697_110000/RConn2
  _CN_88191017_110000_CN_174431697_110000/RConn3 -- T_174431697__Devonport_Substation/LConn3 -- bus40/LConn1
  T_175174348__/LConn1 -- _CN_88191017_110000_CN_175174348_110000/RConn1
  T_175174348__/LConn2 -- _CN_88191017_110000_CN_175174348_110000/RConn2
  _CN_88191017_110000_CN_175174348_110000/RConn3 -- T_175174348__/LConn3 -- bus41/LConn1
  _CN_88191017_110000_CN_167791635_110000/RConn1 -- T_167791635__Burnie_Substation/RConn1 -- L_167791635/LConn1
  _CN_88191017_110000_CN_167791635_110000/RConn2 -- T_167791635__Burnie_Substation/RConn2 -- L_167791635/LConn2
  _CN_88191017_110000_CN_167791635_110000/RConn3 -- T_167791635__Burnie_Substation/RConn3 -- L_167791635/LConn3 -- bus42/LConn1
  T_46339655__/LConn1 -- _CN_46339655_110000_CN_46099414_110000/LConn1
  T_46339655__/LConn2 -- _CN_46339655_110000_CN_46099414_110000/LConn2
  _CN_46339655_110000_CN_46099414_110000/LConn3 -- T_46339655__/LConn3 -- bus43/LConn1
  _CN_46339655_110000_CN_46099414_110000/RConn1 -- T_46099414__Loganlea_Substation/RConn1 -- L_46099414/LConn1
  _CN_46339655_110000_CN_46099414_110000/RConn2 -- T_46099414__Loganlea_Substation/RConn2 -- L_46099414/LConn2
  _CN_46339655_110000_CN_46099414_110000/RConn3 -- T_46099414__Loganlea_Substation/RConn3 -- L_46099414/LConn3 -- bus44/LConn1
  _CN_171575468_110000_CN_172878761_110000/RConn1 -- T_172878761__Middle_Ridge_Substation/RConn1 -- _CN_172878761_110000_CN_308160585_110000/RConn1 -- L_172878761/LConn1 -- _CN_172878761_110000_CN_173094501_110000/LConn1
  _CN_171575468_110000_CN_172878761_110000/RConn2 -- T_172878761__Middle_Ridge_Substation/RConn2 -- _CN_172878761_110000_CN_308160585_110000/RConn2 -- L_172878761/LConn2 -- _CN_172878761_110000_CN_173094501_110000/LConn2
  _CN_171575468_110000_CN_172878761_110000/RConn3 -- T_172878761__Middle_Ridge_Substation/RConn3 -- _CN_172878761_110000_CN_308160585_110000/RConn3 -- L_172878761/LConn3 -- bus45/LConn1 -- _CN_172878761_110000_CN_173094501_110000/LConn3
  T_258723245__/LConn1 -- _CN_258723245_110000_CN_168385464_110000/LConn1
  T_258723245__/LConn2 -- _CN_258723245_110000_CN_168385464_110000/LConn2
  _CN_258723245_110000_CN_168385464_110000/LConn3 -- T_258723245__/LConn3 -- bus46/LConn1
  T_168385464__/LConn1 -- _CN_258723245_110000_CN_168385464_110000/RConn1
  T_168385464__/LConn2 -- _CN_258723245_110000_CN_168385464_110000/RConn2
  _CN_258723245_110000_CN_168385464_110000/RConn3 -- T_168385464__/LConn3 -- bus47/LConn1
  _CN_435794582_110000_CN_176275951_110000/RConn1 -- T_176275951__/LConn1 -- _CN_176275951_110000_CN_88199376_110000/LConn1
  _CN_435794582_110000_CN_176275951_110000/RConn2 -- T_176275951__/LConn2 -- _CN_176275951_110000_CN_88199376_110000/LConn2
  _CN_435794582_110000_CN_176275951_110000/RConn3 -- T_176275951__/LConn3 -- _CN_176275951_110000_CN_88199376_110000/LConn3 -- bus48/LConn1
  T_173094501__South_Toowoomba/LConn1 -- _CN_172878761_110000_CN_173094501_110000/RConn1
  T_173094501__South_Toowoomba/LConn2 -- _CN_172878761_110000_CN_173094501_110000/RConn2
  _CN_172878761_110000_CN_173094501_110000/RConn3 -- T_173094501__South_Toowoomba/LConn3 -- bus49/LConn1
  T_19388978__Rocklea_Substation/LConn1 -- _CN_19388978_110000_CN_302351763_110000/LConn1
  T_19388978__Rocklea_Substation/LConn2 -- _CN_19388978_110000_CN_302351763_110000/LConn2
  _CN_19388978_110000_CN_302351763_110000/LConn3 -- T_19388978__Rocklea_Substation/LConn3 -- bus50/LConn1
  T_302351763__Archerfield_Substation/LConn1 -- _CN_19388978_110000_CN_302351763_110000/RConn1
  T_302351763__Archerfield_Substation/LConn2 -- _CN_19388978_110000_CN_302351763_110000/RConn2
  _CN_19388978_110000_CN_302351763_110000/RConn3 -- T_302351763__Archerfield_Substation/LConn3 -- bus51/LConn1
  T_175927476__/LConn1 -- _CN_175927476_110000_CN_175926345_110000/LConn1
  T_175927476__/LConn2 -- _CN_175927476_110000_CN_175926345_110000/LConn2
  _CN_175927476_110000_CN_175926345_110000/LConn3 -- T_175927476__/LConn3 -- bus52/LConn1
  _CN_175927476_110000_CN_175926345_110000/RConn1 -- T_175926345__New_Norfolk_Substation/LConn1 -- _CN_175926345_110000_CN_175926350_110000/RConn1
  _CN_175927476_110000_CN_175926345_110000/RConn2 -- T_175926345__New_Norfolk_Substation/LConn2 -- _CN_175926345_110000_CN_175926350_110000/RConn2
  _CN_175927476_110000_CN_175926345_110000/RConn3 -- T_175926345__New_Norfolk_Substation/LConn3 -- _CN_175926345_110000_CN_175926350_110000/RConn3 -- bus53/LConn1
  _CN_95612087_110000_CN_125600603_110000/LConn1 -- T_95612087__/RConn1 -- L_95612087/LConn1
  _CN_95612087_110000_CN_125600603_110000/LConn2 -- T_95612087__/RConn2 -- L_95612087/LConn2
  _CN_95612087_110000_CN_125600603_110000/LConn3 -- T_95612087__/RConn3 -- L_95612087/LConn3 -- bus54/LConn1
  _CN_95612087_110000_CN_125600603_110000/RConn1 -- T_125600603__Robina_Substation/LConn1 -- _CN_45020488_110000_CN_125600603_110000/LConn1
  _CN_95612087_110000_CN_125600603_110000/RConn2 -- T_125600603__Robina_Substation/LConn2 -- _CN_45020488_110000_CN_125600603_110000/LConn2
  _CN_95612087_110000_CN_125600603_110000/RConn3 -- T_125600603__Robina_Substation/LConn3 -- _CN_45020488_110000_CN_125600603_110000/LConn3 -- bus55/LConn1
  T_30471365__/LConn1 -- _CN_30471365_110000_CN_48853232_110000/LConn1
  T_30471365__/LConn2 -- _CN_30471365_110000_CN_48853232_110000/LConn2
  _CN_30471365_110000_CN_48853232_110000/LConn3 -- T_30471365__/LConn3 -- bus56/LConn1
  T_48853232__/LConn1 -- _CN_30471365_110000_CN_48853232_110000/RConn1
  T_48853232__/LConn2 -- _CN_30471365_110000_CN_48853232_110000/RConn2
  _CN_30471365_110000_CN_48853232_110000/RConn3 -- T_48853232__/LConn3 -- bus57/LConn1
  _CN_45020488_110000_CN_171581686_110000/LConn1 -- T_45020488__Mudgeeraba_Substation/RConn1 -- _CN_45020488_110000_CN_125600603_110000/RConn1 -- L_45020488/LConn1
  _CN_45020488_110000_CN_171581686_110000/LConn2 -- T_45020488__Mudgeeraba_Substation/RConn2 -- _CN_45020488_110000_CN_125600603_110000/RConn2 -- L_45020488/LConn2
  _CN_45020488_110000_CN_171581686_110000/LConn3 -- T_45020488__Mudgeeraba_Substation/RConn3 -- _CN_45020488_110000_CN_125600603_110000/RConn3 -- L_45020488/LConn3 -- bus58/LConn1
  T_171581686__/LConn1 -- _CN_45020488_110000_CN_171581686_110000/RConn1
  T_171581686__/LConn2 -- _CN_45020488_110000_CN_171581686_110000/RConn2
  _CN_45020488_110000_CN_171581686_110000/RConn3 -- T_171581686__/LConn3 -- bus59/LConn1
  T_307100131__/LConn1 -- _CN_307100131_110000_CN_155682345_110000/LConn1
  T_307100131__/LConn2 -- _CN_307100131_110000_CN_155682345_110000/LConn2
  _CN_307100131_110000_CN_155682345_110000/LConn3 -- T_307100131__/LConn3 -- bus60/LConn1
  T_155682345__Stradbroke_Island_Substation/LConn1 -- _CN_307100131_110000_CN_155682345_110000/RConn1
  T_155682345__Stradbroke_Island_Substation/LConn2 -- _CN_307100131_110000_CN_155682345_110000/RConn2
  _CN_307100131_110000_CN_155682345_110000/RConn3 -- T_155682345__Stradbroke_Island_Substation/LConn3 -- bus61/LConn1
  T_234083565__/LConn1 -- Burnie___Waratah_CN_234083164_110000_CN_234083565_110000/RConn1
  T_234083565__/LConn2 -- Burnie___Waratah_CN_234083164_110000_CN_234083565_110000/RConn2
  Burnie___Waratah_CN_234083164_110000_CN_234083565_110000/RConn3 -- T_234083565__/LConn3 -- bus62/LConn1
  G_88199376_/RConn1 -- _CN_176275951_110000_CN_88199376_110000/RConn1
  G_88199376_/RConn2 -- _CN_176275951_110000_CN_88199376_110000/RConn2
  _CN_176275951_110000_CN_88199376_110000/RConn3 -- G_88199376_/RConn3 -- bus63/LConn1
  T_234863481__/LConn1 -- _CN_234863481_110000_CN_234864299_110000/LConn1
  T_234863481__/LConn2 -- _CN_234863481_110000_CN_234864299_110000/LConn2
  _CN_234863481_110000_CN_234864299_110000/LConn3 -- T_234863481__/LConn3 -- bus64/LConn1
  G_234864299_/RConn1 -- _CN_234863481_110000_CN_234864299_110000/RConn1
  G_234864299_/RConn2 -- _CN_234863481_110000_CN_234864299_110000/RConn2
  _CN_234863481_110000_CN_234864299_110000/RConn3 -- G_234864299_/RConn3 -- bus65/LConn1
  T_234176499__/LConn1 -- _CN_234176499_110000_CN_207655859_110000/LConn1
  T_234176499__/LConn2 -- _CN_234176499_110000_CN_207655859_110000/LConn2
  _CN_234176499_110000_CN_207655859_110000/LConn3 -- T_234176499__/LConn3 -- bus66/LConn1
  G_207655859_/RConn1 -- _CN_234176499_110000_CN_207655859_110000/RConn1
  G_207655859_/RConn2 -- _CN_234176499_110000_CN_207655859_110000/RConn2
  _CN_234176499_110000_CN_207655859_110000/RConn3 -- G_207655859_/RConn3 -- bus67/LConn1
  _CN_99848705_132000_CN_173730623_132000/LConn1 -- T_99848705_330000_Tamworth_330_132_subtransmission_substation/RConn1 -- _CN_99848705_132000_CN_366327501_132000/LConn1 -- L_99848705/LConn1
  _CN_99848705_132000_CN_173730623_132000/LConn2 -- T_99848705_330000_Tamworth_330_132_subtransmission_substation/RConn2 -- _CN_99848705_132000_CN_366327501_132000/LConn2 -- L_99848705/LConn2
  _CN_99848705_132000_CN_173730623_132000/LConn3 -- T_99848705_330000_Tamworth_330_132_subtransmission_substation/RConn3 -- _CN_99848705_132000_CN_366327501_132000/LConn3 -- L_99848705/LConn3 -- bus68/LConn1
  T_173730623_132000_Tamworth_132_66_subtransmission_substation/LConn1 -- _CN_99848705_132000_CN_173730623_132000/RConn1
  T_173730623_132000_Tamworth_132_66_subtransmission_substation/LConn2 -- _CN_99848705_132000_CN_173730623_132000/RConn2
  _CN_99848705_132000_CN_173730623_132000/RConn3 -- T_173730623_132000_Tamworth_132_66_subtransmission_substation/LConn3 -- bus69/LConn1
  T_366327501_132000_Gunnedah_subtransmission_substation/LConn1 -- _CN_99848705_132000_CN_366327501_132000/RConn1
  T_366327501_132000_Gunnedah_subtransmission_substation/LConn2 -- _CN_99848705_132000_CN_366327501_132000/RConn2
  _CN_99848705_132000_CN_366327501_132000/RConn3 -- T_366327501_132000_Gunnedah_subtransmission_substation/LConn3 -- bus70/LConn1
  _CN_171582472_132000_CN_171582471_132000/LConn1 -- T_171582472__/LConn1 -- _CN_171582472_132000_CN_171588475_132000/LConn1
  _CN_171582472_132000_CN_171582471_132000/LConn2 -- T_171582472__/LConn2 -- _CN_171582472_132000_CN_171588475_132000/LConn2
  _CN_171582472_132000_CN_171582471_132000/LConn3 -- T_171582472__/LConn3 -- _CN_171582472_132000_CN_171588475_132000/LConn3 -- bus71/LConn1
  G_171582471_Condamine_Power_Station/RConn1 -- _CN_171582472_132000_CN_171582471_132000/RConn1
  G_171582471_Condamine_Power_Station/RConn2 -- _CN_171582472_132000_CN_171582471_132000/RConn2
  _CN_171582472_132000_CN_171582471_132000/RConn3 -- G_171582471_Condamine_Power_Station/RConn3 -- bus72/LConn1
  T_171588475__Chinchilla_Substation/LConn1 -- _CN_171582472_132000_CN_171588475_132000/RConn1
  T_171588475__Chinchilla_Substation/LConn2 -- _CN_171582472_132000_CN_171588475_132000/RConn2
  _CN_171582472_132000_CN_171588475_132000/RConn3 -- T_171588475__Chinchilla_Substation/LConn3 -- bus73/LConn1
  _CN_196363948_132000_CN_194550809_132000/LConn1 -- T_196363948__/RConn1 -- _CN_196363948_132000_CN_194550807_132000/LConn1 -- _CN_196363948_132000_CN_189021048_132000/LConn1 -- _CN_196363948_132000_CN_173224446_132000/LConn1 -- _CN_196363948_132000_CN_173224184_132000/LConn1 -- _CN_196363948_132000_CN_196583888_132000/LConn1 -- _CN_196363948_132000_CN_196020053_132000/LConn1 -- L_196363948/LConn1
  _CN_196363948_132000_CN_194550809_132000/LConn2 -- T_196363948__/RConn2 -- _CN_196363948_132000_CN_194550807_132000/LConn2 -- _CN_196363948_132000_CN_189021048_132000/LConn2 -- _CN_196363948_132000_CN_173224446_132000/LConn2 -- _CN_196363948_132000_CN_173224184_132000/LConn2 -- _CN_196363948_132000_CN_196583888_132000/LConn2 -- _CN_196363948_132000_CN_196020053_132000/LConn2 -- L_196363948/LConn2
  _CN_196363948_132000_CN_194550809_132000/LConn3 -- T_196363948__/RConn3 -- _CN_196363948_132000_CN_194550807_132000/LConn3 -- _CN_196363948_132000_CN_189021048_132000/LConn3 -- _CN_196363948_132000_CN_173224446_132000/LConn3 -- _CN_196363948_132000_CN_173224184_132000/LConn3 -- _CN_196363948_132000_CN_196583888_132000/LConn3 -- _CN_196363948_132000_CN_196020053_132000/LConn3 -- L_196363948/LConn3 -- bus74/LConn1
  T_194550809__/LConn1 -- _CN_196363948_132000_CN_194550809_132000/RConn1
  T_194550809__/LConn2 -- _CN_196363948_132000_CN_194550809_132000/RConn2
  _CN_196363948_132000_CN_194550809_132000/RConn3 -- T_194550809__/LConn3 -- bus75/LConn1
  T_194550807__/LConn1 -- _CN_196363948_132000_CN_194550807_132000/RConn1
  T_194550807__/LConn2 -- _CN_196363948_132000_CN_194550807_132000/RConn2
  _CN_196363948_132000_CN_194550807_132000/RConn3 -- T_194550807__/LConn3 -- bus76/LConn1
  _CN_196363948_132000_CN_189021048_132000/RConn1 -- T_189021048__132_kV_Turkinje/LConn1 -- _CN_192518673_132000_CN_189021048_132000/LConn1 -- _CN_189021048_132000_CN_196583889_132000/LConn1
  _CN_196363948_132000_CN_189021048_132000/RConn2 -- T_189021048__132_kV_Turkinje/LConn2 -- _CN_192518673_132000_CN_189021048_132000/LConn2 -- _CN_189021048_132000_CN_196583889_132000/LConn2
  _CN_196363948_132000_CN_189021048_132000/RConn3 -- T_189021048__132_kV_Turkinje/LConn3 -- _CN_192518673_132000_CN_189021048_132000/LConn3 -- _CN_189021048_132000_CN_196583889_132000/LConn3 -- bus77/LConn1
  T_173224446_132000_132_kV_Innisfail/LConn1 -- _CN_196363948_132000_CN_173224446_132000/RConn1
  T_173224446_132000_132_kV_Innisfail/LConn2 -- _CN_196363948_132000_CN_173224446_132000/RConn2
  _CN_196363948_132000_CN_173224446_132000/RConn3 -- T_173224446_132000_132_kV_Innisfail/LConn3 -- bus78/LConn1
  T_173224184_132000_132_kV_El_Arish/LConn1 -- _CN_196363948_132000_CN_173224184_132000/RConn1
  T_173224184_132000_132_kV_El_Arish/LConn2 -- _CN_196363948_132000_CN_173224184_132000/RConn2
  _CN_196363948_132000_CN_173224184_132000/RConn3 -- T_173224184_132000_132_kV_El_Arish/LConn3 -- bus79/LConn1
  _CN_196363948_132000_CN_196583888_132000/RConn1 -- T_196583888_132000_132_kV_Tully/LConn1 -- _CN_196583887_132000_CN_196583888_132000/LConn1
  _CN_196363948_132000_CN_196583888_132000/RConn2 -- T_196583888_132000_132_kV_Tully/LConn2 -- _CN_196583887_132000_CN_196583888_132000/LConn2
  _CN_196363948_132000_CN_196583888_132000/RConn3 -- T_196583888_132000_132_kV_Tully/LConn3 -- _CN_196583887_132000_CN_196583888_132000/LConn3 -- bus80/LConn1
  T_196020053_132000_132_kV_Edmonton/LConn1 -- _CN_196363948_132000_CN_196020053_132000/RConn1
  T_196020053_132000_132_kV_Edmonton/LConn2 -- _CN_196363948_132000_CN_196020053_132000/RConn2
  _CN_196363948_132000_CN_196020053_132000/RConn3 -- T_196020053_132000_132_kV_Edmonton/LConn3 -- bus81/LConn1
  T_173396697__/LConn1 -- _CN_173396697_132000_CN_169406848_132000/LConn1
  T_173396697__/LConn2 -- _CN_173396697_132000_CN_169406848_132000/LConn2
  _CN_173396697_132000_CN_169406848_132000/LConn3 -- T_173396697__/LConn3 -- bus82/LConn1
  _CN_173396697_132000_CN_169406848_132000/RConn1 -- T_169406848__Wellington_substation/RConn1 -- _CN_169406848_132000_CN_174991765_132000/LConn1 -- L_169406848/LConn1
  _CN_173396697_132000_CN_169406848_132000/RConn2 -- T_169406848__Wellington_substation/RConn2 -- _CN_169406848_132000_CN_174991765_132000/LConn2 -- L_169406848/LConn2
  _CN_173396697_132000_CN_169406848_132000/RConn3 -- T_169406848__Wellington_substation/RConn3 -- _CN_169406848_132000_CN_174991765_132000/LConn3 -- L_169406848/LConn3 -- bus83/LConn1
  T_205012494__/LConn1 -- _CN_205012494_132000_CN_205012488_132000/LConn1
  T_205012494__/LConn2 -- _CN_205012494_132000_CN_205012488_132000/LConn2
  _CN_205012494_132000_CN_205012488_132000/LConn3 -- T_205012494__/LConn3 -- bus84/LConn1
  T_205012488__/LConn1 -- _CN_205012494_132000_CN_205012488_132000/RConn1
  T_205012488__/LConn2 -- _CN_205012494_132000_CN_205012488_132000/RConn2
  _CN_205012494_132000_CN_205012488_132000/RConn3 -- T_205012488__/LConn3 -- bus85/LConn1
  _CN_119871505_132000_CN_344076960_132000/LConn1 -- T_119871505__/RConn1 -- _CN_119871505_132000_CN_160191425_132000/LConn1 -- _CN_119871505_132000_CN_174036841_132000/LConn1 -- L_119871505/LConn1
  _CN_119871505_132000_CN_344076960_132000/LConn2 -- T_119871505__/RConn2 -- _CN_119871505_132000_CN_160191425_132000/LConn2 -- _CN_119871505_132000_CN_174036841_132000/LConn2 -- L_119871505/LConn2
  _CN_119871505_132000_CN_344076960_132000/LConn3 -- T_119871505__/RConn3 -- _CN_119871505_132000_CN_160191425_132000/LConn3 -- _CN_119871505_132000_CN_174036841_132000/LConn3 -- L_119871505/LConn3 -- bus86/LConn1
  T_344076960__/LConn1 -- _CN_119871505_132000_CN_344076960_132000/RConn1
  T_344076960__/LConn2 -- _CN_119871505_132000_CN_344076960_132000/RConn2
  _CN_119871505_132000_CN_344076960_132000/RConn3 -- T_344076960__/LConn3 -- bus87/LConn1
  _CN_119871505_132000_CN_160191425_132000/RConn1 -- T_160191425__/RConn1 -- _CN_163374875_132000_CN_160191425_132000/LConn1 -- _CN_163374877_132000_CN_160191425_132000/LConn1 -- _CN_166192455_132000_CN_160191425_132000/LConn1 -- L_160191425/LConn1
  _CN_119871505_132000_CN_160191425_132000/RConn2 -- T_160191425__/RConn2 -- _CN_163374875_132000_CN_160191425_132000/LConn2 -- _CN_163374877_132000_CN_160191425_132000/LConn2 -- _CN_166192455_132000_CN_160191425_132000/LConn2 -- L_160191425/LConn2
  _CN_119871505_132000_CN_160191425_132000/RConn3 -- T_160191425__/RConn3 -- _CN_163374875_132000_CN_160191425_132000/LConn3 -- _CN_163374877_132000_CN_160191425_132000/LConn3 -- _CN_166192455_132000_CN_160191425_132000/LConn3 -- L_160191425/LConn3 -- bus88/LConn1
  T_174036841__Cowra_substation/LConn1 -- _CN_119871505_132000_CN_174036841_132000/RConn1
  T_174036841__Cowra_substation/LConn2 -- _CN_119871505_132000_CN_174036841_132000/RConn2
  _CN_119871505_132000_CN_174036841_132000/RConn3 -- T_174036841__Cowra_substation/LConn3 -- bus89/LConn1
  _CN_214977199_132000_CN_166192455_132000/LConn1 -- T_214977199__/LConn1 -- _CN_214977199_132000_CN_163374878_132000/LConn1
  _CN_214977199_132000_CN_166192455_132000/LConn2 -- T_214977199__/LConn2 -- _CN_214977199_132000_CN_163374878_132000/LConn2
  _CN_214977199_132000_CN_166192455_132000/LConn3 -- T_214977199__/LConn3 -- _CN_214977199_132000_CN_163374878_132000/LConn3 -- bus90/LConn1
  _CN_214977199_132000_CN_166192455_132000/RConn1 -- T_166192455__/LConn1 -- _CN_166192455_132000_CN_160191425_132000/RConn1
  _CN_214977199_132000_CN_166192455_132000/RConn2 -- T_166192455__/LConn2 -- _CN_166192455_132000_CN_160191425_132000/RConn2
  _CN_214977199_132000_CN_166192455_132000/RConn3 -- T_166192455__/LConn3 -- _CN_166192455_132000_CN_160191425_132000/RConn3 -- bus91/LConn1
  _CN_214977199_132000_CN_163374878_132000/RConn1 -- T_163374878__Bruce_Substation/LConn1 -- _CN_163374878_132000_CN_163374879_132000/LConn1
  _CN_214977199_132000_CN_163374878_132000/RConn2 -- T_163374878__Bruce_Substation/LConn2 -- _CN_163374878_132000_CN_163374879_132000/LConn2
  _CN_214977199_132000_CN_163374878_132000/RConn3 -- T_163374878__Bruce_Substation/LConn3 -- _CN_163374878_132000_CN_163374879_132000/LConn3 -- bus92/LConn1
  T_192353822_132000;66000;22000_Lakeland_Substation/LConn1 -- _CN_192353822_132000_CN_191779550_132000/LConn1
  T_192353822_132000;66000;22000_Lakeland_Substation/LConn2 -- _CN_192353822_132000_CN_191779550_132000/LConn2
  _CN_192353822_132000_CN_191779550_132000/LConn3 -- T_192353822_132000;66000;22000_Lakeland_Substation/LConn3 -- bus93/LConn1
  _CN_192353822_132000_CN_191779550_132000/RConn1 -- T_191779550__/LConn1 -- _CN_192518673_132000_CN_191779550_132000/LConn1
  _CN_192353822_132000_CN_191779550_132000/RConn2 -- T_191779550__/LConn2 -- _CN_192518673_132000_CN_191779550_132000/LConn2
  _CN_192353822_132000_CN_191779550_132000/RConn3 -- T_191779550__/LConn3 -- _CN_192518673_132000_CN_191779550_132000/LConn3 -- bus94/LConn1
  T_232106017__/LConn1 -- _CN_232106017_132000_CN_232109241_132000/LConn1
  T_232106017__/LConn2 -- _CN_232106017_132000_CN_232109241_132000/LConn2
  _CN_232106017_132000_CN_232109241_132000/LConn3 -- T_232106017__/LConn3 -- bus95/LConn1
  _CN_232106017_132000_CN_232109241_132000/RConn1 -- T_232109241__Williamsdale/LConn1 -- _CN_439689405_132000_CN_232109241_132000/LConn1
  _CN_232106017_132000_CN_232109241_132000/RConn2 -- T_232109241__Williamsdale/LConn2 -- _CN_439689405_132000_CN_232109241_132000/LConn2
  _CN_232106017_132000_CN_232109241_132000/RConn3 -- T_232109241__Williamsdale/LConn3 -- _CN_439689405_132000_CN_232109241_132000/LConn3 -- bus96/LConn1
  T_172230182__/LConn1 -- _CN_172230182_132000_CN_172231145_132000/LConn1
  T_172230182__/LConn2 -- _CN_172230182_132000_CN_172231145_132000/LConn2
  _CN_172230182_132000_CN_172231145_132000/LConn3 -- T_172230182__/LConn3 -- bus97/LConn1
  _CN_172230182_132000_CN_172231145_132000/RConn1 -- T_172231145__/RConn1 -- _CN_174246471_132000_CN_172231145_132000/LConn1 -- L_172231145/LConn1
  _CN_172230182_132000_CN_172231145_132000/RConn2 -- T_172231145__/RConn2 -- _CN_174246471_132000_CN_172231145_132000/LConn2 -- L_172231145/LConn2
  _CN_172230182_132000_CN_172231145_132000/RConn3 -- T_172231145__/RConn3 -- _CN_174246471_132000_CN_172231145_132000/LConn3 -- L_172231145/LConn3 -- bus98/LConn1
  _CN_234539007_132000_CN_160201298_132000/LConn1 -- T_234539007__Glen_Innes_subtransmission_station/LConn1 -- _CN_234539007_132000_CN_340560031_132000/LConn1
  _CN_234539007_132000_CN_160201298_132000/LConn2 -- T_234539007__Glen_Innes_subtransmission_station/LConn2 -- _CN_234539007_132000_CN_340560031_132000/LConn2
  _CN_234539007_132000_CN_160201298_132000/LConn3 -- T_234539007__Glen_Innes_subtransmission_station/LConn3 -- _CN_234539007_132000_CN_340560031_132000/LConn3 -- bus99/LConn1
  _CN_234539007_132000_CN_160201298_132000/RConn1 -- T_160201298__Armidale_Substation/RConn1 -- _CN_160201298_132000_CN_171962240_132000/LConn1 -- _CN_160201298_132000_CN_172891041_132000/LConn1 -- L_160201298/LConn1
  _CN_234539007_132000_CN_160201298_132000/RConn2 -- T_160201298__Armidale_Substation/RConn2 -- _CN_160201298_132000_CN_171962240_132000/LConn2 -- _CN_160201298_132000_CN_172891041_132000/LConn2 -- L_160201298/LConn2
  _CN_234539007_132000_CN_160201298_132000/RConn3 -- T_160201298__Armidale_Substation/RConn3 -- _CN_160201298_132000_CN_171962240_132000/LConn3 -- _CN_160201298_132000_CN_172891041_132000/LConn3 -- L_160201298/LConn3 -- bus100/LConn1
  T_340560031__Tenterfield_subtransmission_station/LConn1 -- _CN_234539007_132000_CN_340560031_132000/RConn1
  T_340560031__Tenterfield_subtransmission_station/LConn2 -- _CN_234539007_132000_CN_340560031_132000/RConn2
  _CN_234539007_132000_CN_340560031_132000/RConn3 -- T_340560031__Tenterfield_subtransmission_station/LConn3 -- bus101/LConn1
  _CN_179921457_132000_CN_175862605_132000/LConn1 -- T_179921457__Belrose_Substation/LConn1 -- _CN_179921457_132000_CN_45727589_132000/LConn1 -- _CN_179921457_132000_CN_179923658_132000/LConn1
  _CN_179921457_132000_CN_175862605_132000/LConn2 -- T_179921457__Belrose_Substation/LConn2 -- _CN_179921457_132000_CN_45727589_132000/LConn2 -- _CN_179921457_132000_CN_179923658_132000/LConn2
  _CN_179921457_132000_CN_175862605_132000/LConn3 -- T_179921457__Belrose_Substation/LConn3 -- _CN_179921457_132000_CN_45727589_132000/LConn3 -- bus102/LConn1 -- _CN_179921457_132000_CN_179923658_132000/LConn3
  _CN_179921457_132000_CN_175862605_132000/RConn1 -- T_175862605__/LConn1 -- _CN_284934380_132000_CN_175862605_132000/LConn1
  _CN_179921457_132000_CN_175862605_132000/RConn2 -- T_175862605__/LConn2 -- _CN_284934380_132000_CN_175862605_132000/LConn2
  _CN_179921457_132000_CN_175862605_132000/RConn3 -- T_175862605__/LConn3 -- _CN_284934380_132000_CN_175862605_132000/LConn3 -- bus103/LConn1
  _CN_179921457_132000_CN_179923658_132000/RConn1 -- T_179923658__/RConn1 -- _CN_174124088_132000_CN_179923658_132000/LConn1 -- L_179923658/LConn1
  _CN_179921457_132000_CN_179923658_132000/RConn2 -- T_179923658__/RConn2 -- _CN_174124088_132000_CN_179923658_132000/LConn2 -- L_179923658/LConn2
  _CN_179921457_132000_CN_179923658_132000/RConn3 -- T_179923658__/RConn3 -- _CN_174124088_132000_CN_179923658_132000/LConn3 -- L_179923658/LConn3 -- bus104/LConn1
  _CN_179921457_132000_CN_45727589_132000/RConn1 -- T_45727589__/LConn1 -- _CN_45727591_132000_CN_45727589_132000/LConn1
  _CN_179921457_132000_CN_45727589_132000/RConn2 -- T_45727589__/LConn2 -- _CN_45727591_132000_CN_45727589_132000/LConn2
  _CN_179921457_132000_CN_45727589_132000/RConn3 -- T_45727589__/LConn3 -- _CN_45727591_132000_CN_45727589_132000/LConn3 -- bus105/LConn1
  T_224223242__/LConn1 -- _CN_224223242_132000_CN_44192327_132000/LConn1
  T_224223242__/LConn2 -- _CN_224223242_132000_CN_44192327_132000/LConn2
  _CN_224223242_132000_CN_44192327_132000/LConn3 -- T_224223242__/LConn3 -- bus106/LConn1
  T_44192327__/LConn1 -- _CN_224223242_132000_CN_44192327_132000/RConn1
  T_44192327__/LConn2 -- _CN_224223242_132000_CN_44192327_132000/RConn2
  _CN_224223242_132000_CN_44192327_132000/RConn3 -- T_44192327__/LConn3 -- bus107/LConn1
  _CN_164764211_132000_CN_169687537_132000/LConn1 -- T_164764211__/LConn1 -- _CN_164764211_132000_CN_164675939_132000/LConn1
  _CN_164764211_132000_CN_169687537_132000/LConn2 -- T_164764211__/LConn2 -- _CN_164764211_132000_CN_164675939_132000/LConn2
  _CN_164764211_132000_CN_169687537_132000/LConn3 -- T_164764211__/LConn3 -- _CN_164764211_132000_CN_164675939_132000/LConn3 -- bus108/LConn1
  T_169687537__Keith_substation/LConn1 -- _CN_164764211_132000_CN_169687537_132000/RConn1
  T_169687537__Keith_substation/LConn2 -- _CN_164764211_132000_CN_169687537_132000/RConn2
  _CN_164764211_132000_CN_169687537_132000/RConn3 -- T_169687537__Keith_substation/LConn3 -- bus109/LConn1
  _CN_164764211_132000_CN_164675939_132000/RConn1 -- T_164675939__ElectraNet_South_East_Substation/RConn1 -- _CN_164682851_132000_CN_164675939_132000/LConn1 -- L_164675939/LConn1
  _CN_164764211_132000_CN_164675939_132000/RConn2 -- T_164675939__ElectraNet_South_East_Substation/RConn2 -- _CN_164682851_132000_CN_164675939_132000/LConn2 -- L_164675939/LConn2
  _CN_164764211_132000_CN_164675939_132000/RConn3 -- T_164675939__ElectraNet_South_East_Substation/RConn3 -- _CN_164682851_132000_CN_164675939_132000/LConn3 -- L_164675939/LConn3 -- bus110/LConn1
  _CN_267376693_132000_CN_267376695_132000/LConn1 -- T_267376693__Bateman's_Bay/LConn1 -- _CN_267376693_132000_CN_267376701_132000/LConn1
  _CN_267376693_132000_CN_267376695_132000/LConn2 -- T_267376693__Bateman's_Bay/LConn2 -- _CN_267376693_132000_CN_267376701_132000/LConn2
  _CN_267376693_132000_CN_267376695_132000/LConn3 -- T_267376693__Bateman's_Bay/LConn3 -- _CN_267376693_132000_CN_267376701_132000/LConn3 -- bus111/LConn1
  _CN_267376693_132000_CN_267376695_132000/RConn1 -- T_267376695__Evans_Lane_Zone_Substation/LConn1 -- _CN_267376695_132000_CN_267376699_132000/LConn1 -- _CN_267376695_132000_CN_267376698_132000/LConn1 -- _CN_267376695_132000_CN_267376701_132000/LConn1
  _CN_267376693_132000_CN_267376695_132000/RConn2 -- T_267376695__Evans_Lane_Zone_Substation/LConn2 -- _CN_267376695_132000_CN_267376699_132000/LConn2 -- _CN_267376695_132000_CN_267376698_132000/LConn2 -- _CN_267376695_132000_CN_267376701_132000/LConn2
  _CN_267376693_132000_CN_267376695_132000/RConn3 -- T_267376695__Evans_Lane_Zone_Substation/LConn3 -- _CN_267376695_132000_CN_267376699_132000/LConn3 -- _CN_267376695_132000_CN_267376698_132000/LConn3 -- _CN_267376695_132000_CN_267376701_132000/LConn3 -- bus112/LConn1
  _CN_267376693_132000_CN_267376701_132000/RConn1 -- T_267376701__/LConn1 -- _CN_267376695_132000_CN_267376701_132000/RConn1
  _CN_267376693_132000_CN_267376701_132000/RConn2 -- T_267376701__/LConn2 -- _CN_267376695_132000_CN_267376701_132000/RConn2
  _CN_267376693_132000_CN_267376701_132000/RConn3 -- T_267376701__/LConn3 -- _CN_267376695_132000_CN_267376701_132000/RConn3 -- bus113/LConn1
  _CN_173102134_132000_CN_174835009_132000/LConn1 -- T_173102134__/RConn1 -- _CN_173102134_132000_CN_174831245_132000/LConn1 -- L_173102134/LConn1
  _CN_173102134_132000_CN_174835009_132000/LConn2 -- T_173102134__/RConn2 -- _CN_173102134_132000_CN_174831245_132000/LConn2 -- L_173102134/LConn2
  _CN_173102134_132000_CN_174835009_132000/LConn3 -- T_173102134__/RConn3 -- _CN_173102134_132000_CN_174831245_132000/LConn3 -- L_173102134/LConn3 -- bus114/LConn1
  _CN_173102134_132000_CN_174835009_132000/RConn1 -- T_174835009__/LConn1 -- _CN_174831245_132000_CN_174835009_132000/LConn1
  _CN_173102134_132000_CN_174835009_132000/RConn2 -- T_174835009__/LConn2 -- _CN_174831245_132000_CN_174835009_132000/LConn2
  _CN_173102134_132000_CN_174835009_132000/RConn3 -- T_174835009__/LConn3 -- _CN_174831245_132000_CN_174835009_132000/LConn3 -- bus115/LConn1
  _CN_173102134_132000_CN_174831245_132000/RConn1 -- T_174831245__/LConn1 -- _CN_174831245_132000_CN_108712269_132000/LConn1 -- _CN_174831245_132000_CN_174835009_132000/RConn1 -- _CN_174831245_132000_CN_50334999_132000/LConn1
  _CN_173102134_132000_CN_174831245_132000/RConn2 -- T_174831245__/LConn2 -- _CN_174831245_132000_CN_108712269_132000/LConn2 -- _CN_174831245_132000_CN_174835009_132000/RConn2 -- _CN_174831245_132000_CN_50334999_132000/LConn2
  _CN_173102134_132000_CN_174831245_132000/RConn3 -- T_174831245__/LConn3 -- _CN_174831245_132000_CN_108712269_132000/LConn3 -- _CN_174831245_132000_CN_174835009_132000/RConn3 -- bus116/LConn1 -- _CN_174831245_132000_CN_50334999_132000/LConn3
  T_267376699__Ulladulla_Zone_Substation/LConn1 -- _CN_267376695_132000_CN_267376699_132000/RConn1
  T_267376699__Ulladulla_Zone_Substation/LConn2 -- _CN_267376695_132000_CN_267376699_132000/RConn2
  _CN_267376695_132000_CN_267376699_132000/RConn3 -- T_267376699__Ulladulla_Zone_Substation/LConn3 -- bus117/LConn1
  _CN_267376695_132000_CN_267376698_132000/RConn1 -- T_267376698_132000;33000_Shoalhaven_Transmission_Substation/LConn1 -- _CN_255998100_132000_CN_267376698_132000/LConn1
  _CN_267376695_132000_CN_267376698_132000/RConn2 -- T_267376698_132000;33000_Shoalhaven_Transmission_Substation/LConn2 -- _CN_255998100_132000_CN_267376698_132000/LConn2
  _CN_267376695_132000_CN_267376698_132000/RConn3 -- T_267376698_132000;33000_Shoalhaven_Transmission_Substation/LConn3 -- _CN_255998100_132000_CN_267376698_132000/LConn3 -- bus118/LConn1
  T_174124088__/LConn1 -- _CN_174124088_132000_CN_179923658_132000/RConn1
  T_174124088__/LConn2 -- _CN_174124088_132000_CN_179923658_132000/RConn2
  _CN_174124088_132000_CN_179923658_132000/RConn3 -- T_174124088__/LConn3 -- bus119/LConn1
  T_171746362__/LConn1 -- _CN_171746362_132000_CN_171744984_132000/LConn1
  T_171746362__/LConn2 -- _CN_171746362_132000_CN_171744984_132000/LConn2
  _CN_171746362_132000_CN_171744984_132000/LConn3 -- T_171746362__/LConn3 -- bus120/LConn1
  T_171744984__/LConn1 -- _CN_171746362_132000_CN_171744984_132000/RConn1
  T_171744984__/LConn2 -- _CN_171746362_132000_CN_171744984_132000/RConn2
  _CN_171746362_132000_CN_171744984_132000/RConn3 -- T_171744984__/LConn3 -- bus121/LConn1
  _CN_366321212_132000_CN_172891041_132000/LConn1 -- T_366321212_132000_Moree_subtransmission_substation/LConn1 -- _CN_366321212_132000_CN_366605305_132000/LConn1
  _CN_366321212_132000_CN_172891041_132000/LConn2 -- T_366321212_132000_Moree_subtransmission_substation/LConn2 -- _CN_366321212_132000_CN_366605305_132000/LConn2
  _CN_366321212_132000_CN_172891041_132000/LConn3 -- T_366321212_132000_Moree_subtransmission_substation/LConn3 -- _CN_366321212_132000_CN_366605305_132000/LConn3 -- bus122/LConn1
  _CN_366321212_132000_CN_172891041_132000/RConn1 -- T_172891041__Inverell_subtransmission_station/LConn1 -- _CN_160201298_132000_CN_172891041_132000/RConn1
  _CN_366321212_132000_CN_172891041_132000/RConn2 -- T_172891041__Inverell_subtransmission_station/LConn2 -- _CN_160201298_132000_CN_172891041_132000/RConn2
  _CN_366321212_132000_CN_172891041_132000/RConn3 -- T_172891041__Inverell_subtransmission_station/LConn3 -- _CN_160201298_132000_CN_172891041_132000/RConn3 -- bus123/LConn1
  T_366605305_132000_Narrabri_subtransmission_substation/LConn1 -- _CN_366321212_132000_CN_366605305_132000/RConn1
  T_366605305_132000_Narrabri_subtransmission_substation/LConn2 -- _CN_366321212_132000_CN_366605305_132000/RConn2
  _CN_366321212_132000_CN_366605305_132000/RConn3 -- T_366605305_132000_Narrabri_subtransmission_substation/LConn3 -- bus124/LConn1
  _CN_47069245_132000_CN_45402899_132000/LConn1 -- T_47069245__Mount_Lawley_sub_station/LConn1 -- _CN_47069245_132000_CN_145689826_132000/LConn1 -- _CN_47069245_132000_CN_44187488_132000/LConn1
  _CN_47069245_132000_CN_45402899_132000/LConn2 -- T_47069245__Mount_Lawley_sub_station/LConn2 -- _CN_47069245_132000_CN_145689826_132000/LConn2 -- _CN_47069245_132000_CN_44187488_132000/LConn2
  _CN_47069245_132000_CN_45402899_132000/LConn3 -- T_47069245__Mount_Lawley_sub_station/LConn3 -- _CN_47069245_132000_CN_145689826_132000/LConn3 -- _CN_47069245_132000_CN_44187488_132000/LConn3 -- bus125/LConn1
  T_45402899__/LConn1 -- _CN_47069245_132000_CN_45402899_132000/RConn1
  T_45402899__/LConn2 -- _CN_47069245_132000_CN_45402899_132000/RConn2
  _CN_47069245_132000_CN_45402899_132000/RConn3 -- T_45402899__/LConn3 -- bus126/LConn1
  T_145689826__/LConn1 -- _CN_47069245_132000_CN_145689826_132000/RConn1
  T_145689826__/LConn2 -- _CN_47069245_132000_CN_145689826_132000/RConn2
  _CN_47069245_132000_CN_145689826_132000/RConn3 -- T_145689826__/LConn3 -- bus127/LConn1
  _CN_47069245_132000_CN_44187488_132000/RConn1 -- T_44187488__/RConn1 -- _CN_44140812_132000_CN_44187488_132000/LConn1 -- _CN_44187488_132000_CN_46503657_132000/LConn1 -- L_44187488/LConn1
  _CN_47069245_132000_CN_44187488_132000/RConn2 -- T_44187488__/RConn2 -- _CN_44140812_132000_CN_44187488_132000/LConn2 -- _CN_44187488_132000_CN_46503657_132000/LConn2 -- L_44187488/LConn2
  _CN_47069245_132000_CN_44187488_132000/RConn3 -- T_44187488__/RConn3 -- _CN_44140812_132000_CN_44187488_132000/LConn3 -- _CN_44187488_132000_CN_46503657_132000/LConn3 -- L_44187488/LConn3 -- bus128/LConn1
  _CN_171852863_132000_CN_72231236_132000/LConn1 -- T_171852863__/LConn1 -- _CN_171852863_132000_CN_170990862_132000/LConn1
  _CN_171852863_132000_CN_72231236_132000/LConn2 -- T_171852863__/LConn2 -- _CN_171852863_132000_CN_170990862_132000/LConn2
  _CN_171852863_132000_CN_72231236_132000/LConn3 -- T_171852863__/LConn3 -- _CN_171852863_132000_CN_170990862_132000/LConn3 -- bus129/LConn1
  _CN_171852863_132000_CN_72231236_132000/RConn1 -- T_72231236__/LConn1 -- _CN_83991232_132000_CN_72231236_132000/LConn1 -- _CN_72231242_132000_CN_72231236_132000/LConn1
  _CN_171852863_132000_CN_72231236_132000/RConn2 -- T_72231236__/LConn2 -- _CN_83991232_132000_CN_72231236_132000/LConn2 -- _CN_72231242_132000_CN_72231236_132000/LConn2
  _CN_171852863_132000_CN_72231236_132000/RConn3 -- T_72231236__/LConn3 -- _CN_83991232_132000_CN_72231236_132000/LConn3 -- _CN_72231242_132000_CN_72231236_132000/LConn3 -- bus130/LConn1
  _CN_171852863_132000_CN_170990862_132000/RConn1 -- T_170990862__/RConn1 -- _CN_170990862_132000_CN_171734315_132000/LConn1 -- L_170990862/LConn1
  _CN_171852863_132000_CN_170990862_132000/RConn2 -- T_170990862__/RConn2 -- _CN_170990862_132000_CN_171734315_132000/LConn2 -- L_170990862/LConn2
  _CN_171852863_132000_CN_170990862_132000/RConn3 -- T_170990862__/RConn3 -- _CN_170990862_132000_CN_171734315_132000/LConn3 -- L_170990862/LConn3 -- bus131/LConn1
  T_312679496__Macarthur_Wind_Farm_Substation/LConn1 -- _CN_312679496_132000_CN_312551365_132000/LConn1
  T_312679496__Macarthur_Wind_Farm_Substation/LConn2 -- _CN_312679496_132000_CN_312551365_132000/LConn2
  _CN_312679496_132000_CN_312551365_132000/LConn3 -- T_312679496__Macarthur_Wind_Farm_Substation/LConn3 -- bus132/LConn1
  _CN_312679496_132000_CN_312551365_132000/RConn1 -- T_312551365__/LConn1 -- _CN_312551544_132000_CN_312551365_132000/LConn1
  _CN_312679496_132000_CN_312551365_132000/RConn2 -- T_312551365__/LConn2 -- _CN_312551544_132000_CN_312551365_132000/LConn2
  _CN_312679496_132000_CN_312551365_132000/RConn3 -- T_312551365__/LConn3 -- _CN_312551544_132000_CN_312551365_132000/LConn3 -- bus133/LConn1
  T_48579657__/LConn1 -- _CN_48579657_132000_CN_133353043_132000/LConn1
  T_48579657__/LConn2 -- _CN_48579657_132000_CN_133353043_132000/LConn2
  _CN_48579657_132000_CN_133353043_132000/LConn3 -- T_48579657__/LConn3 -- bus134/LConn1
  _CN_48579657_132000_CN_133353043_132000/RConn1 -- T_133353043__/LConn1 -- _CN_133353043_132000_CN_44140812_132000/LConn1 -- _CN_133353043_132000_CN_214229754_132000/LConn1
  _CN_48579657_132000_CN_133353043_132000/RConn2 -- T_133353043__/LConn2 -- _CN_133353043_132000_CN_44140812_132000/LConn2 -- _CN_133353043_132000_CN_214229754_132000/LConn2
  _CN_48579657_132000_CN_133353043_132000/RConn3 -- T_133353043__/LConn3 -- _CN_133353043_132000_CN_44140812_132000/LConn3 -- _CN_133353043_132000_CN_214229754_132000/LConn3 -- bus135/LConn1
  T_47036496__/LConn1 -- _CN_47036496_132000_CN_175920440_132000/LConn1
  T_47036496__/LConn2 -- _CN_47036496_132000_CN_175920440_132000/LConn2
  _CN_47036496_132000_CN_175920440_132000/LConn3 -- T_47036496__/LConn3 -- bus136/LConn1
  _CN_47036496_132000_CN_175920440_132000/RConn1 -- T_175920440__Sydney_South/RConn1 -- _CN_175920440_132000_CN_218450415_132000/LConn1 -- L_175920440/LConn1
  _CN_47036496_132000_CN_175920440_132000/RConn2 -- T_175920440__Sydney_South/RConn2 -- _CN_175920440_132000_CN_218450415_132000/LConn2 -- L_175920440/LConn2
  _CN_47036496_132000_CN_175920440_132000/RConn3 -- T_175920440__Sydney_South/RConn3 -- _CN_175920440_132000_CN_218450415_132000/LConn3 -- L_175920440/LConn3 -- bus137/LConn1
  _CN_45553233_132000_CN_37106603_132000/LConn1 -- T_45553233__/RConn1 -- L_45553233/LConn1
  _CN_45553233_132000_CN_37106603_132000/LConn2 -- T_45553233__/RConn2 -- L_45553233/LConn2
  _CN_45553233_132000_CN_37106603_132000/LConn3 -- T_45553233__/RConn3 -- L_45553233/LConn3 -- bus138/LConn1
  T_37106603__/LConn1 -- _CN_45553233_132000_CN_37106603_132000/RConn1
  T_37106603__/LConn2 -- _CN_45553233_132000_CN_37106603_132000/RConn2
  _CN_45553233_132000_CN_37106603_132000/RConn3 -- T_37106603__/LConn3 -- bus139/LConn1
  _CN_160201298_132000_CN_171962240_132000/RConn1 -- T_171962240_132000_Koolkhan_subtransmission_substation/LConn1 -- _CN_171962240_132000_CN_171581408_132000/LConn1
  _CN_160201298_132000_CN_171962240_132000/RConn2 -- T_171962240_132000_Koolkhan_subtransmission_substation/LConn2 -- _CN_171962240_132000_CN_171581408_132000/LConn2
  _CN_160201298_132000_CN_171962240_132000/RConn3 -- T_171962240_132000_Koolkhan_subtransmission_substation/LConn3 -- _CN_171962240_132000_CN_171581408_132000/LConn3 -- bus140/LConn1
  _CN_133353043_132000_CN_44140812_132000/RConn1 -- T_44140812__/LConn1 -- _CN_44140812_132000_CN_44187488_132000/RConn1
  _CN_133353043_132000_CN_44140812_132000/RConn2 -- T_44140812__/LConn2 -- _CN_44140812_132000_CN_44187488_132000/RConn2
  _CN_133353043_132000_CN_44140812_132000/RConn3 -- T_44140812__/LConn3 -- _CN_44140812_132000_CN_44187488_132000/RConn3 -- bus141/LConn1
  T_214229754__/LConn1 -- _CN_133353043_132000_CN_214229754_132000/RConn1
  T_214229754__/LConn2 -- _CN_133353043_132000_CN_214229754_132000/RConn2
  _CN_133353043_132000_CN_214229754_132000/RConn3 -- T_214229754__/LConn3 -- bus142/LConn1
  T_231510030__/LConn1 -- _CN_231510030_132000_CN_170066302_132000/LConn1
  T_231510030__/LConn2 -- _CN_231510030_132000_CN_170066302_132000/LConn2
  _CN_231510030_132000_CN_170066302_132000/LConn3 -- T_231510030__/LConn3 -- bus143/LConn1
  T_170066302__/LConn1 -- _CN_231510030_132000_CN_170066302_132000/RConn1
  T_170066302__/LConn2 -- _CN_231510030_132000_CN_170066302_132000/RConn2
  _CN_231510030_132000_CN_170066302_132000/RConn3 -- T_170066302__/LConn3 -- bus144/LConn1
  T_239698383__/LConn1 -- _CN_239698383_132000_CN_24028364_132000/LConn1
  T_239698383__/LConn2 -- _CN_239698383_132000_CN_24028364_132000/LConn2
  _CN_239698383_132000_CN_24028364_132000/LConn3 -- T_239698383__/LConn3 -- bus145/LConn1
  _CN_239698383_132000_CN_24028364_132000/RConn1 -- T_24028364__Newcastle_substation/RConn1 -- _CN_24028364_132000_CN_242555644_132000/LConn1 -- L_24028364/LConn1
  _CN_239698383_132000_CN_24028364_132000/RConn2 -- T_24028364__Newcastle_substation/RConn2 -- _CN_24028364_132000_CN_242555644_132000/LConn2 -- L_24028364/LConn2
  _CN_239698383_132000_CN_24028364_132000/RConn3 -- T_24028364__Newcastle_substation/RConn3 -- _CN_24028364_132000_CN_242555644_132000/LConn3 -- L_24028364/LConn3 -- bus146/LConn1
  T_167924823__/LConn1 -- _CN_167924823_132000_CN_165154628_132000/LConn1
  T_167924823__/LConn2 -- _CN_167924823_132000_CN_165154628_132000/LConn2
  _CN_167924823_132000_CN_165154628_132000/LConn3 -- T_167924823__/LConn3 -- bus147/LConn1
  _CN_167924823_132000_CN_165154628_132000/RConn1 -- T_165154628__/RConn1 -- L_165154628/LConn1
  _CN_167924823_132000_CN_165154628_132000/RConn2 -- T_165154628__/RConn2 -- L_165154628/LConn2
  _CN_167924823_132000_CN_165154628_132000/RConn3 -- T_165154628__/RConn3 -- L_165154628/LConn3 -- bus148/LConn1
  T_224939099__Kewdale_sub_station/LConn1 -- _CN_224939099_132000_CN_224958207_132000/LConn1
  T_224939099__Kewdale_sub_station/LConn2 -- _CN_224939099_132000_CN_224958207_132000/LConn2
  _CN_224939099_132000_CN_224958207_132000/LConn3 -- T_224939099__Kewdale_sub_station/LConn3 -- bus149/LConn1
  _CN_224939099_132000_CN_224958207_132000/RConn1 -- T_224958207__Belmont_sub_station/LConn1 -- _CN_224945355_132000_CN_224958207_132000/LConn1
  _CN_224939099_132000_CN_224958207_132000/RConn2 -- T_224958207__Belmont_sub_station/LConn2 -- _CN_224945355_132000_CN_224958207_132000/LConn2
  _CN_224939099_132000_CN_224958207_132000/RConn3 -- T_224958207__Belmont_sub_station/LConn3 -- _CN_224945355_132000_CN_224958207_132000/LConn3 -- bus150/LConn1
  T_165170273__/LConn1 -- _CN_165170273_132000_CN_165169360_132000/LConn1
  T_165170273__/LConn2 -- _CN_165170273_132000_CN_165169360_132000/LConn2
  _CN_165170273_132000_CN_165169360_132000/LConn3 -- T_165170273__/LConn3 -- bus151/LConn1
  T_165169360__/LConn1 -- _CN_165170273_132000_CN_165169360_132000/RConn1
  T_165169360__/LConn2 -- _CN_165170273_132000_CN_165169360_132000/RConn2
  _CN_165170273_132000_CN_165169360_132000/RConn3 -- T_165169360__/LConn3 -- bus152/LConn1
  _CN_171582050_132000_CN_170840487_132000/LConn1 -- T_171582050__Mooloolaba_Substation/LConn1 -- _CN_171582050_132000_CN_328503276_132000/LConn1
  _CN_171582050_132000_CN_170840487_132000/LConn2 -- T_171582050__Mooloolaba_Substation/LConn2 -- _CN_171582050_132000_CN_328503276_132000/LConn2
  _CN_171582050_132000_CN_170840487_132000/LConn3 -- T_171582050__Mooloolaba_Substation/LConn3 -- _CN_171582050_132000_CN_328503276_132000/LConn3 -- bus153/LConn1
  _CN_171582050_132000_CN_170840487_132000/RConn1 -- T_170840487__Palmwoods_Substation/LConn1 -- _CN_72231242_132000_CN_170840487_132000/LConn1
  _CN_171582050_132000_CN_170840487_132000/RConn2 -- T_170840487__Palmwoods_Substation/LConn2 -- _CN_72231242_132000_CN_170840487_132000/LConn2
  _CN_171582050_132000_CN_170840487_132000/RConn3 -- T_170840487__Palmwoods_Substation/LConn3 -- _CN_72231242_132000_CN_170840487_132000/LConn3 -- bus154/LConn1
  T_328503276__Alexandra_Headlands_Substation/LConn1 -- _CN_171582050_132000_CN_328503276_132000/RConn1
  T_328503276__Alexandra_Headlands_Substation/LConn2 -- _CN_171582050_132000_CN_328503276_132000/RConn2
  _CN_171582050_132000_CN_328503276_132000/RConn3 -- T_328503276__Alexandra_Headlands_Substation/LConn3 -- bus155/LConn1
  T_164682851__/LConn1 -- _CN_164682851_132000_CN_164675939_132000/RConn1
  T_164682851__/LConn2 -- _CN_164682851_132000_CN_164675939_132000/RConn2
  _CN_164682851_132000_CN_164675939_132000/RConn3 -- T_164682851__/LConn3 -- bus156/LConn1
  _CN_192518673_132000_CN_191779550_132000/RConn1 -- T_192518673__Craiglie_132kV_Substation/LConn1 -- _CN_192518673_132000_CN_189021048_132000/RConn1
  _CN_192518673_132000_CN_191779550_132000/RConn2 -- T_192518673__Craiglie_132kV_Substation/LConn2 -- _CN_192518673_132000_CN_189021048_132000/RConn2
  _CN_192518673_132000_CN_191779550_132000/RConn3 -- T_192518673__Craiglie_132kV_Substation/LConn3 -- _CN_192518673_132000_CN_189021048_132000/RConn3 -- bus157/LConn1
  _CN_171735144_132000_CN_173551375_132000/LConn1 -- T_171735144__/LConn1 -- _CN_171735144_132000_CN_171002668_132000/LConn1 -- _CN_171735144_132000_CN_171734315_132000/LConn1
  _CN_171735144_132000_CN_173551375_132000/LConn2 -- T_171735144__/LConn2 -- _CN_171735144_132000_CN_171002668_132000/LConn2 -- _CN_171735144_132000_CN_171734315_132000/LConn2
  _CN_171735144_132000_CN_173551375_132000/LConn3 -- T_171735144__/LConn3 -- _CN_171735144_132000_CN_171002668_132000/LConn3 -- _CN_171735144_132000_CN_171734315_132000/LConn3 -- bus158/LConn1
  _CN_171735144_132000_CN_173551375_132000/RConn1 -- T_173551375__Isis_substation/LConn1 -- _CN_173551375_132000_CN_175017770_132000/LConn1
  _CN_171735144_132000_CN_173551375_132000/RConn2 -- T_173551375__Isis_substation/LConn2 -- _CN_173551375_132000_CN_175017770_132000/LConn2
  _CN_171735144_132000_CN_173551375_132000/RConn3 -- T_173551375__Isis_substation/LConn3 -- _CN_173551375_132000_CN_175017770_132000/LConn3 -- bus159/LConn1
  _CN_171735144_132000_CN_171002668_132000/RConn1 -- T_171002668__/RConn1 -- L_171002668/LConn1
  _CN_171735144_132000_CN_171002668_132000/RConn2 -- T_171002668__/RConn2 -- L_171002668/LConn2
  _CN_171735144_132000_CN_171002668_132000/RConn3 -- T_171002668__/RConn3 -- L_171002668/LConn3 -- bus160/LConn1
  _CN_171735144_132000_CN_171734315_132000/RConn1 -- T_171734315__Kilkivan_Substation/LConn1 -- _CN_170990862_132000_CN_171734315_132000/RConn1
  _CN_171735144_132000_CN_171734315_132000/RConn2 -- T_171734315__Kilkivan_Substation/LConn2 -- _CN_170990862_132000_CN_171734315_132000/RConn2
  _CN_171735144_132000_CN_171734315_132000/RConn3 -- T_171734315__Kilkivan_Substation/LConn3 -- _CN_170990862_132000_CN_171734315_132000/RConn3 -- bus161/LConn1
  T_45727591__/LConn1 -- _CN_45727591_132000_CN_45727589_132000/RConn1
  T_45727591__/LConn2 -- _CN_45727591_132000_CN_45727589_132000/RConn2
  _CN_45727591_132000_CN_45727589_132000/RConn3 -- T_45727591__/LConn3 -- bus162/LConn1
  T_439689405_132000_Cooma/LConn1 -- _CN_439689405_132000_CN_232109241_132000/RConn1
  T_439689405_132000_Cooma/LConn2 -- _CN_439689405_132000_CN_232109241_132000/RConn2
  _CN_439689405_132000_CN_232109241_132000/RConn3 -- T_439689405_132000_Cooma/LConn3 -- bus163/LConn1
  T_121671797__Transgrid_Port_Macquarie_Substation/LConn1 -- _CN_121671797_132000_CN_205011577_132000/LConn1
  T_121671797__Transgrid_Port_Macquarie_Substation/LConn2 -- _CN_121671797_132000_CN_205011577_132000/LConn2
  _CN_121671797_132000_CN_205011577_132000/LConn3 -- T_121671797__Transgrid_Port_Macquarie_Substation/LConn3 -- bus164/LConn1
  T_205011577_132000_Kempsey_subtransmission_substation/LConn1 -- _CN_121671797_132000_CN_205011577_132000/RConn1
  T_205011577_132000_Kempsey_subtransmission_substation/LConn2 -- _CN_121671797_132000_CN_205011577_132000/RConn2
  _CN_121671797_132000_CN_205011577_132000/RConn3 -- T_205011577_132000_Kempsey_subtransmission_substation/LConn3 -- bus165/LConn1
  T_312551544__/LConn1 -- _CN_312551544_132000_CN_312551365_132000/RConn1
  T_312551544__/LConn2 -- _CN_312551544_132000_CN_312551365_132000/RConn2
  _CN_312551544_132000_CN_312551365_132000/RConn3 -- T_312551544__/LConn3 -- bus166/LConn1
  T_69034090__/LConn1 -- _CN_69034090_132000_CN_54674751_132000/LConn1
  T_69034090__/LConn2 -- _CN_69034090_132000_CN_54674751_132000/LConn2
  _CN_69034090_132000_CN_54674751_132000/LConn3 -- T_69034090__/LConn3 -- bus167/LConn1
  _CN_69034090_132000_CN_54674751_132000/RConn1 -- T_54674751__Gladstone_Power_Station_Sub_Station/RConn1 -- _CN_54674751_132000_CN_432510474_132000/LConn1 -- L_54674751/LConn1
  _CN_69034090_132000_CN_54674751_132000/RConn2 -- T_54674751__Gladstone_Power_Station_Sub_Station/RConn2 -- _CN_54674751_132000_CN_432510474_132000/LConn2 -- L_54674751/LConn2
  _CN_69034090_132000_CN_54674751_132000/RConn3 -- T_54674751__Gladstone_Power_Station_Sub_Station/RConn3 -- _CN_54674751_132000_CN_432510474_132000/LConn3 -- L_54674751/LConn3 -- bus168/LConn1
  _CN_254440062_132000_CN_161829167_132000/LConn1 -- T_254440062__/LConn1 -- _CN_254440062_132000_CN_165712061_132000/LConn1
  _CN_254440062_132000_CN_161829167_132000/LConn2 -- T_254440062__/LConn2 -- _CN_254440062_132000_CN_165712061_132000/LConn2
  _CN_254440062_132000_CN_161829167_132000/LConn3 -- T_254440062__/LConn3 -- _CN_254440062_132000_CN_165712061_132000/LConn3 -- bus169/LConn1
  _CN_254440062_132000_CN_161829167_132000/RConn1 -- T_161829167__Ourimbah_Substation/LConn1 -- _CN_161829167_132000_CN_165709781_132000/LConn1
  _CN_254440062_132000_CN_161829167_132000/RConn2 -- T_161829167__Ourimbah_Substation/LConn2 -- _CN_161829167_132000_CN_165709781_132000/LConn2
  _CN_254440062_132000_CN_161829167_132000/RConn3 -- T_161829167__Ourimbah_Substation/LConn3 -- _CN_161829167_132000_CN_165709781_132000/LConn3 -- bus170/LConn1
  T_165712061__/LConn1 -- _CN_254440062_132000_CN_165712061_132000/RConn1
  T_165712061__/LConn2 -- _CN_254440062_132000_CN_165712061_132000/RConn2
  _CN_254440062_132000_CN_165712061_132000/RConn3 -- T_165712061__/LConn3 -- bus171/LConn1
  252_Hornsby___Berowra_CN_179068556_132000_CN_178929982_132000/LConn1 -- T_179068556__Hornsby_Substation/LConn1 -- Hornsby___Pennant_Hills_132kV_CN_179068556_132000_CN_179085999_132000/LConn1
  252_Hornsby___Berowra_CN_179068556_132000_CN_178929982_132000/LConn2 -- T_179068556__Hornsby_Substation/LConn2 -- Hornsby___Pennant_Hills_132kV_CN_179068556_132000_CN_179085999_132000/LConn2
  252_Hornsby___Berowra_CN_179068556_132000_CN_178929982_132000/LConn3 -- T_179068556__Hornsby_Substation/LConn3 -- Hornsby___Pennant_Hills_132kV_CN_179068556_132000_CN_179085999_132000/LConn3 -- bus172/LConn1
  T_178929982__/LConn1 -- 252_Hornsby___Berowra_CN_179068556_132000_CN_178929982_132000/RConn1
  T_178929982__/LConn2 -- 252_Hornsby___Berowra_CN_179068556_132000_CN_178929982_132000/RConn2
  252_Hornsby___Berowra_CN_179068556_132000_CN_178929982_132000/RConn3 -- T_178929982__/LConn3 -- bus173/LConn1
  T_179085999__/LConn1 -- Hornsby___Pennant_Hills_132kV_CN_179068556_132000_CN_179085999_132000/RConn1
  T_179085999__/LConn2 -- Hornsby___Pennant_Hills_132kV_CN_179068556_132000_CN_179085999_132000/RConn2
  Hornsby___Pennant_Hills_132kV_CN_179068556_132000_CN_179085999_132000/RConn3 -- T_179085999__/LConn3 -- bus174/LConn1
  T_50334999__Transgrid_Mulwala_Substation/LConn1 -- _CN_174831245_132000_CN_50334999_132000/RConn1
  T_50334999__Transgrid_Mulwala_Substation/LConn2 -- _CN_174831245_132000_CN_50334999_132000/RConn2
  _CN_174831245_132000_CN_50334999_132000/RConn3 -- T_50334999__Transgrid_Mulwala_Substation/LConn3 -- bus175/LConn1
  T_108712269__/LConn1 -- _CN_174831245_132000_CN_108712269_132000/RConn1
  T_108712269__/LConn2 -- _CN_174831245_132000_CN_108712269_132000/RConn2
  _CN_174831245_132000_CN_108712269_132000/RConn3 -- T_108712269__/LConn3 -- bus176/LConn1
  _CN_255998100_132000_CN_172620016_132000/LConn1 -- T_255998100_132000;33000_Mount_Terry_Transmission_Substation/LConn1 -- _CN_255998100_132000_CN_267376698_132000/RConn1
  _CN_255998100_132000_CN_172620016_132000/LConn2 -- T_255998100_132000;33000_Mount_Terry_Transmission_Substation/LConn2 -- _CN_255998100_132000_CN_267376698_132000/RConn2
  _CN_255998100_132000_CN_172620016_132000/LConn3 -- T_255998100_132000;33000_Mount_Terry_Transmission_Substation/LConn3 -- _CN_255998100_132000_CN_267376698_132000/RConn3 -- bus177/LConn1
  _CN_255998100_132000_CN_172620016_132000/RConn1 -- T_172620016_330000;132000_Dapto_Transmission_Substation/RConn1 -- _CN_172620016_132000_CN_255775145_132000/LConn1 -- _CN_172620016_132000_CN_227898159_132000/LConn1 -- _CN_172620016_132000_CN_142733661_132000/LConn1 -- L_172620016/LConn1
  _CN_255998100_132000_CN_172620016_132000/RConn2 -- T_172620016_330000;132000_Dapto_Transmission_Substation/RConn2 -- _CN_172620016_132000_CN_255775145_132000/LConn2 -- _CN_172620016_132000_CN_227898159_132000/LConn2 -- _CN_172620016_132000_CN_142733661_132000/LConn2 -- L_172620016/LConn2
  _CN_255998100_132000_CN_172620016_132000/RConn3 -- T_172620016_330000;132000_Dapto_Transmission_Substation/RConn3 -- _CN_172620016_132000_CN_255775145_132000/LConn3 -- _CN_172620016_132000_CN_227898159_132000/LConn3 -- _CN_172620016_132000_CN_142733661_132000/LConn3 -- L_172620016/LConn3 -- bus178/LConn1
  T_239285915__/LConn1 -- _CN_239285915_132000_CN_166089888_132000/LConn1
  T_239285915__/LConn2 -- _CN_239285915_132000_CN_166089888_132000/LConn2
  _CN_239285915_132000_CN_166089888_132000/LConn3 -- T_239285915__/LConn3 -- bus179/LConn1
  T_166089888__Beresfield_Substransmission_Substation/LConn1 -- _CN_239285915_132000_CN_166089888_132000/RConn1
  T_166089888__Beresfield_Substransmission_Substation/LConn2 -- _CN_239285915_132000_CN_166089888_132000/RConn2
  _CN_239285915_132000_CN_166089888_132000/RConn3 -- T_166089888__Beresfield_Substransmission_Substation/LConn3 -- bus180/LConn1
  T_255998114__BOC_Substation/LConn1 -- _CN_255998114_132000_CN_142733661_132000/LConn1
  T_255998114__BOC_Substation/LConn2 -- _CN_255998114_132000_CN_142733661_132000/LConn2
  _CN_255998114_132000_CN_142733661_132000/LConn3 -- T_255998114__BOC_Substation/LConn3 -- bus181/LConn1
  _CN_255998114_132000_CN_142733661_132000/RConn1 -- T_142733661_132000;33000_Springhill_Transmission_Substation/LConn1 -- _CN_142733661_132000_CN_255775145_132000/LConn1 -- _CN_142733661_132000_CN_255775138_132000/LConn1 -- _CN_172620016_132000_CN_142733661_132000/RConn1
  _CN_255998114_132000_CN_142733661_132000/RConn2 -- T_142733661_132000;33000_Springhill_Transmission_Substation/LConn2 -- _CN_142733661_132000_CN_255775145_132000/LConn2 -- _CN_142733661_132000_CN_255775138_132000/LConn2 -- _CN_172620016_132000_CN_142733661_132000/RConn2
  _CN_255998114_132000_CN_142733661_132000/RConn3 -- T_142733661_132000;33000_Springhill_Transmission_Substation/LConn3 -- _CN_142733661_132000_CN_255775145_132000/LConn3 -- bus182/LConn1 -- _CN_142733661_132000_CN_255775138_132000/LConn3 -- _CN_172620016_132000_CN_142733661_132000/RConn3
  _CN_174246471_132000_CN_363077936_132000/LConn1 -- T_174246471__/LConn1 -- _CN_174246471_132000_CN_172231145_132000/RConn1 -- _CN_174246471_132000_CN_174246481_132000/LConn1 -- _CN_174246471_132000_CN_180773850_132000/LConn1
  _CN_174246471_132000_CN_363077936_132000/LConn2 -- T_174246471__/LConn2 -- _CN_174246471_132000_CN_172231145_132000/RConn2 -- _CN_174246471_132000_CN_174246481_132000/LConn2 -- _CN_174246471_132000_CN_180773850_132000/LConn2
  _CN_174246471_132000_CN_363077936_132000/LConn3 -- T_174246471__/LConn3 -- _CN_174246471_132000_CN_172231145_132000/RConn3 -- _CN_174246471_132000_CN_174246481_132000/LConn3 -- _CN_174246471_132000_CN_180773850_132000/LConn3 -- bus183/LConn1
  T_363077936_132000_/LConn1 -- _CN_174246471_132000_CN_363077936_132000/RConn1
  T_363077936_132000_/LConn2 -- _CN_174246471_132000_CN_363077936_132000/RConn2
  _CN_174246471_132000_CN_363077936_132000/RConn3 -- T_363077936_132000_/LConn3 -- bus184/LConn1
  T_174246481__/LConn1 -- _CN_174246471_132000_CN_174246481_132000/RConn1
  T_174246481__/LConn2 -- _CN_174246471_132000_CN_174246481_132000/RConn2
  _CN_174246471_132000_CN_174246481_132000/RConn3 -- T_174246481__/LConn3 -- bus185/LConn1
  T_180773850__/LConn1 -- _CN_174246471_132000_CN_180773850_132000/RConn1
  T_180773850__/LConn2 -- _CN_174246471_132000_CN_180773850_132000/RConn2
  _CN_174246471_132000_CN_180773850_132000/RConn3 -- T_180773850__/LConn3 -- bus186/LConn1
  _CN_160295596_132000_CN_267376696_132000/LConn1 -- T_160295596_330000;132000_Marulan_Transmission_Substation/RConn1 -- L_160295596/LConn1
  _CN_160295596_132000_CN_267376696_132000/LConn2 -- T_160295596_330000;132000_Marulan_Transmission_Substation/RConn2 -- L_160295596/LConn2
  _CN_160295596_132000_CN_267376696_132000/LConn3 -- T_160295596_330000;132000_Marulan_Transmission_Substation/RConn3 -- L_160295596/LConn3 -- bus187/LConn1
  T_267376696_132000;33000_Fairfax_Lane_Transmission_Substation/LConn1 -- _CN_160295596_132000_CN_267376696_132000/RConn1
  T_267376696_132000;33000_Fairfax_Lane_Transmission_Substation/LConn2 -- _CN_160295596_132000_CN_267376696_132000/RConn2
  _CN_160295596_132000_CN_267376696_132000/RConn3 -- T_267376696_132000;33000_Fairfax_Lane_Transmission_Substation/LConn3 -- bus188/LConn1
  _CN_170407602_132000_CN_170407657_132000/LConn1 -- T_170407602__/LConn1 -- _CN_170407602_132000_CN_164764363_132000/LConn1
  _CN_170407602_132000_CN_170407657_132000/LConn2 -- T_170407602__/LConn2 -- _CN_170407602_132000_CN_164764363_132000/LConn2
  _CN_170407602_132000_CN_170407657_132000/LConn3 -- T_170407602__/LConn3 -- _CN_170407602_132000_CN_164764363_132000/LConn3 -- bus189/LConn1
  T_170407657__/LConn1 -- _CN_170407602_132000_CN_170407657_132000/RConn1
  T_170407657__/LConn2 -- _CN_170407602_132000_CN_170407657_132000/RConn2
  _CN_170407602_132000_CN_170407657_132000/RConn3 -- T_170407657__/LConn3 -- bus190/LConn1
  _CN_170407602_132000_CN_164764363_132000/RConn1 -- T_164764363__/RConn1 -- L_164764363/LConn1
  _CN_170407602_132000_CN_164764363_132000/RConn2 -- T_164764363__/RConn2 -- L_164764363/LConn2
  _CN_170407602_132000_CN_164764363_132000/RConn3 -- T_164764363__/RConn3 -- L_164764363/LConn3 -- bus191/LConn1
  T_173401274__/LConn1 -- _CN_173401274_132000_CN_174991765_132000/LConn1
  T_173401274__/LConn2 -- _CN_173401274_132000_CN_174991765_132000/LConn2
  _CN_173401274_132000_CN_174991765_132000/LConn3 -- T_173401274__/LConn3 -- bus192/LConn1
  _CN_173401274_132000_CN_174991765_132000/RConn1 -- T_174991765__/LConn1 -- _CN_169406848_132000_CN_174991765_132000/RConn1
  _CN_173401274_132000_CN_174991765_132000/RConn2 -- T_174991765__/LConn2 -- _CN_169406848_132000_CN_174991765_132000/RConn2
  _CN_173401274_132000_CN_174991765_132000/RConn3 -- T_174991765__/LConn3 -- _CN_169406848_132000_CN_174991765_132000/RConn3 -- bus193/LConn1
  T_83991232__/LConn1 -- _CN_83991232_132000_CN_72231236_132000/RConn1
  T_83991232__/LConn2 -- _CN_83991232_132000_CN_72231236_132000/RConn2
  _CN_83991232_132000_CN_72231236_132000/RConn3 -- T_83991232__/LConn3 -- bus194/LConn1
  _CN_169408193_132000_CN_174239045_132000/LConn1 -- T_169408193__/RConn1 -- L_169408193/LConn1
  _CN_169408193_132000_CN_174239045_132000/LConn2 -- T_169408193__/RConn2 -- L_169408193/LConn2
  _CN_169408193_132000_CN_174239045_132000/LConn3 -- T_169408193__/RConn3 -- L_169408193/LConn3 -- bus195/LConn1
  T_174239045__/LConn1 -- _CN_169408193_132000_CN_174239045_132000/RConn1
  T_174239045__/LConn2 -- _CN_169408193_132000_CN_174239045_132000/RConn2
  _CN_169408193_132000_CN_174239045_132000/RConn3 -- T_174239045__/LConn3 -- bus196/LConn1
  _CN_172245698_132000_CN_171845369_132000/LConn1 -- T_172245698__/LConn1 -- _CN_172245698_132000_CN_172246489_132000/LConn1 -- _CN_172245698_132000_CN_172246523_132000/LConn1
  _CN_172245698_132000_CN_171845369_132000/LConn2 -- T_172245698__/LConn2 -- _CN_172245698_132000_CN_172246489_132000/LConn2 -- _CN_172245698_132000_CN_172246523_132000/LConn2
  _CN_172245698_132000_CN_171845369_132000/LConn3 -- T_172245698__/LConn3 -- _CN_172245698_132000_CN_172246489_132000/LConn3 -- bus197/LConn1 -- _CN_172245698_132000_CN_172246523_132000/LConn3
  _CN_172245698_132000_CN_171845369_132000/RConn1 -- T_171845369__/LConn1 -- _CN_298020591_132000_CN_171845369_132000/LConn1
  _CN_172245698_132000_CN_171845369_132000/RConn2 -- T_171845369__/LConn2 -- _CN_298020591_132000_CN_171845369_132000/LConn2
  _CN_172245698_132000_CN_171845369_132000/RConn3 -- T_171845369__/LConn3 -- _CN_298020591_132000_CN_171845369_132000/LConn3 -- bus198/LConn1
  G_172246523_/RConn1 -- _CN_172245698_132000_CN_172246523_132000/RConn1
  G_172246523_/RConn2 -- _CN_172245698_132000_CN_172246523_132000/RConn2
  _CN_172245698_132000_CN_172246523_132000/RConn3 -- G_172246523_/RConn3 -- bus199/LConn1
  T_172246489__/LConn1 -- _CN_172245698_132000_CN_172246489_132000/RConn1
  T_172246489__/LConn2 -- _CN_172245698_132000_CN_172246489_132000/RConn2
  _CN_172245698_132000_CN_172246489_132000/RConn3 -- T_172246489__/LConn3 -- bus200/LConn1
  T_242555644__/LConn1 -- _CN_24028364_132000_CN_242555644_132000/RConn1
  T_242555644__/LConn2 -- _CN_24028364_132000_CN_242555644_132000/RConn2
  _CN_24028364_132000_CN_242555644_132000/RConn3 -- T_242555644__/LConn3 -- bus201/LConn1
  _CN_164775125_132000_CN_164774384_132000/LConn1 -- T_164775125__/RConn1 -- L_164775125/LConn1
  _CN_164775125_132000_CN_164774384_132000/LConn2 -- T_164775125__/RConn2 -- L_164775125/LConn2
  _CN_164775125_132000_CN_164774384_132000/LConn3 -- T_164775125__/RConn3 -- L_164775125/LConn3 -- bus202/LConn1
  T_164774384__/LConn1 -- _CN_164775125_132000_CN_164774384_132000/RConn1
  T_164774384__/LConn2 -- _CN_164775125_132000_CN_164774384_132000/RConn2
  _CN_164775125_132000_CN_164774384_132000/RConn3 -- T_164774384__/LConn3 -- bus203/LConn1
  _CN_234528471_132000_CN_164025782_132000/LConn1 -- T_234528471__/LConn1 -- _CN_234528471_132000_CN_169416665_132000/LConn1
  _CN_234528471_132000_CN_164025782_132000/LConn2 -- T_234528471__/LConn2 -- _CN_234528471_132000_CN_169416665_132000/LConn2
  _CN_234528471_132000_CN_164025782_132000/LConn3 -- T_234528471__/LConn3 -- _CN_234528471_132000_CN_169416665_132000/LConn3 -- bus204/LConn1
  _CN_234528471_132000_CN_164025782_132000/RConn1 -- T_164025782__/LConn1 -- _CN_164025782_132000_CN_169416665_132000/LConn1
  _CN_234528471_132000_CN_164025782_132000/RConn2 -- T_164025782__/LConn2 -- _CN_164025782_132000_CN_169416665_132000/LConn2
  _CN_234528471_132000_CN_164025782_132000/RConn3 -- T_164025782__/LConn3 -- _CN_164025782_132000_CN_169416665_132000/LConn3 -- bus205/LConn1
  _CN_234528471_132000_CN_169416665_132000/RConn1 -- T_169416665__/RConn1 -- _CN_164025782_132000_CN_169416665_132000/RConn1 -- L_169416665/LConn1
  _CN_234528471_132000_CN_169416665_132000/RConn2 -- T_169416665__/RConn2 -- _CN_164025782_132000_CN_169416665_132000/RConn2 -- L_169416665/LConn2
  _CN_234528471_132000_CN_169416665_132000/RConn3 -- T_169416665__/RConn3 -- _CN_164025782_132000_CN_169416665_132000/RConn3 -- L_169416665/LConn3 -- bus206/LConn1
  _CN_196583887_132000_CN_196583888_132000/RConn1 -- T_196583887_132000_132_kV_Kareeya/LConn1 -- _CN_196583887_132000_CN_196583889_132000/LConn1
  _CN_196583887_132000_CN_196583888_132000/RConn2 -- T_196583887_132000_132_kV_Kareeya/LConn2 -- _CN_196583887_132000_CN_196583889_132000/LConn2
  _CN_196583887_132000_CN_196583888_132000/RConn3 -- T_196583887_132000_132_kV_Kareeya/LConn3 -- _CN_196583887_132000_CN_196583889_132000/LConn3 -- bus207/LConn1
  _CN_196583887_132000_CN_196583889_132000/RConn1 -- T_196583889_275000_275_kV_Chalumbin/RConn1 -- _CN_189021048_132000_CN_196583889_132000/RConn1 -- L_196583889/LConn1
  _CN_196583887_132000_CN_196583889_132000/RConn2 -- T_196583889_275000_275_kV_Chalumbin/RConn2 -- _CN_189021048_132000_CN_196583889_132000/RConn2 -- L_196583889/LConn2
  _CN_196583887_132000_CN_196583889_132000/RConn3 -- T_196583889_275000_275_kV_Chalumbin/RConn3 -- _CN_189021048_132000_CN_196583889_132000/RConn3 -- L_196583889/LConn3 -- bus208/LConn1
  T_172998381__/LConn1 -- _CN_172998381_132000_CN_75514732_132000/LConn1
  T_172998381__/LConn2 -- _CN_172998381_132000_CN_75514732_132000/LConn2
  _CN_172998381_132000_CN_75514732_132000/LConn3 -- T_172998381__/LConn3 -- bus209/LConn1
  _CN_172998381_132000_CN_75514732_132000/RConn1 -- T_75514732__/RConn1 -- L_75514732/LConn1
  _CN_172998381_132000_CN_75514732_132000/RConn2 -- T_75514732__/RConn2 -- L_75514732/LConn2
  _CN_172998381_132000_CN_75514732_132000/RConn3 -- T_75514732__/RConn3 -- L_75514732/LConn3 -- bus210/LConn1
  T_298020591__/LConn1 -- _CN_298020591_132000_CN_171845369_132000/RConn1
  T_298020591__/LConn2 -- _CN_298020591_132000_CN_171845369_132000/RConn2
  _CN_298020591_132000_CN_171845369_132000/RConn3 -- T_298020591__/LConn3 -- bus211/LConn1
  _CN_172620016_132000_CN_255775145_132000/RConn1 -- T_255775145_132000_Tallawarra_Substation/LConn1 -- _CN_142733661_132000_CN_255775145_132000/RConn1
  _CN_172620016_132000_CN_255775145_132000/RConn2 -- T_255775145_132000_Tallawarra_Substation/LConn2 -- _CN_142733661_132000_CN_255775145_132000/RConn2
  _CN_172620016_132000_CN_255775145_132000/RConn3 -- T_255775145_132000_Tallawarra_Substation/LConn3 -- _CN_142733661_132000_CN_255775145_132000/RConn3 -- bus212/LConn1
  T_227898159_132000;33000_Bellambi_Transmission_Substation/LConn1 -- _CN_172620016_132000_CN_227898159_132000/RConn1
  T_227898159_132000;33000_Bellambi_Transmission_Substation/LConn2 -- _CN_172620016_132000_CN_227898159_132000/RConn2
  _CN_172620016_132000_CN_227898159_132000/RConn3 -- T_227898159_132000;33000_Bellambi_Transmission_Substation/LConn3 -- bus213/LConn1
  _CN_224945355_132000_CN_225196539_132000/LConn1 -- T_224945355__/LConn1 -- _CN_224945355_132000_CN_224958207_132000/RConn1
  _CN_224945355_132000_CN_225196539_132000/LConn2 -- T_224945355__/LConn2 -- _CN_224945355_132000_CN_224958207_132000/RConn2
  _CN_224945355_132000_CN_225196539_132000/LConn3 -- T_224945355__/LConn3 -- _CN_224945355_132000_CN_224958207_132000/RConn3 -- bus214/LConn1
  T_225196539__/LConn1 -- _CN_224945355_132000_CN_225196539_132000/RConn1
  T_225196539__/LConn2 -- _CN_224945355_132000_CN_225196539_132000/RConn2
  _CN_224945355_132000_CN_225196539_132000/RConn3 -- T_225196539__/LConn3 -- bus215/LConn1
  T_171581252__/LConn1 -- _CN_171581252_132000_CN_171581408_132000/LConn1
  T_171581252__/LConn2 -- _CN_171581252_132000_CN_171581408_132000/LConn2
  _CN_171581252_132000_CN_171581408_132000/LConn3 -- T_171581252__/LConn3 -- bus216/LConn1
  _CN_171581252_132000_CN_171581408_132000/RConn1 -- T_171581408__Lismore_330_132_subtransmission_station/RConn1 -- _CN_171962240_132000_CN_171581408_132000/RConn1 -- L_171581408/LConn1
  _CN_171581252_132000_CN_171581408_132000/RConn2 -- T_171581408__Lismore_330_132_subtransmission_station/RConn2 -- _CN_171962240_132000_CN_171581408_132000/RConn2 -- L_171581408/LConn2
  _CN_171581252_132000_CN_171581408_132000/RConn3 -- T_171581408__Lismore_330_132_subtransmission_station/RConn3 -- _CN_171962240_132000_CN_171581408_132000/RConn3 -- L_171581408/LConn3 -- bus217/LConn1
  _CN_173551375_132000_CN_175017770_132000/RConn1 -- T_175017770__Bundaberg_substation/LConn1 -- _CN_175017770_132000_CN_175020086_132000/LConn1
  _CN_173551375_132000_CN_175017770_132000/RConn2 -- T_175017770__Bundaberg_substation/LConn2 -- _CN_175017770_132000_CN_175020086_132000/LConn2
  _CN_173551375_132000_CN_175017770_132000/RConn3 -- T_175017770__Bundaberg_substation/LConn3 -- _CN_175017770_132000_CN_175020086_132000/LConn3 -- bus218/LConn1
  _CN_163374875_132000_CN_160191425_132000/RConn1 -- T_163374875__Latham_Substation/LConn1 -- _CN_163374875_132000_CN_163374879_132000/LConn1
  _CN_163374875_132000_CN_160191425_132000/RConn2 -- T_163374875__Latham_Substation/LConn2 -- _CN_163374875_132000_CN_163374879_132000/LConn2
  _CN_163374875_132000_CN_160191425_132000/RConn3 -- T_163374875__Latham_Substation/LConn3 -- _CN_163374875_132000_CN_163374879_132000/LConn3 -- bus219/LConn1
  _CN_163374875_132000_CN_163374879_132000/RConn1 -- T_163374879__Belconnen_Substation/LConn1 -- _CN_163374878_132000_CN_163374879_132000/RConn1
  _CN_163374875_132000_CN_163374879_132000/RConn2 -- T_163374879__Belconnen_Substation/LConn2 -- _CN_163374878_132000_CN_163374879_132000/RConn2
  _CN_163374875_132000_CN_163374879_132000/RConn3 -- T_163374879__Belconnen_Substation/LConn3 -- _CN_163374878_132000_CN_163374879_132000/RConn3 -- bus220/LConn1
  _CN_163374877_132000_CN_166184400_132000/LConn1 -- T_163374877__Gold_Creek_Substation/LConn1 -- _CN_163374877_132000_CN_160191425_132000/RConn1
  _CN_163374877_132000_CN_166184400_132000/LConn2 -- T_163374877__Gold_Creek_Substation/LConn2 -- _CN_163374877_132000_CN_160191425_132000/RConn2
  _CN_163374877_132000_CN_166184400_132000/LConn3 -- T_163374877__Gold_Creek_Substation/LConn3 -- _CN_163374877_132000_CN_160191425_132000/RConn3 -- bus221/LConn1
  _CN_163374877_132000_CN_166184400_132000/RConn1 -- T_166184400__/LConn1 -- _CN_166184400_132000_CN_229813242_132000/LConn1 -- _CN_166184400_132000_CN_229813239_132000/LConn1
  _CN_163374877_132000_CN_166184400_132000/RConn2 -- T_166184400__/LConn2 -- _CN_166184400_132000_CN_229813242_132000/LConn2 -- _CN_166184400_132000_CN_229813239_132000/LConn2
  _CN_163374877_132000_CN_166184400_132000/RConn3 -- T_166184400__/LConn3 -- _CN_166184400_132000_CN_229813242_132000/LConn3 -- _CN_166184400_132000_CN_229813239_132000/LConn3 -- bus222/LConn1
  T_171573029__Biloela_Substation/LConn1 -- _CN_171573029_132000_CN_119996556_132000/LConn1
  T_171573029__Biloela_Substation/LConn2 -- _CN_171573029_132000_CN_119996556_132000/LConn2
  _CN_171573029_132000_CN_119996556_132000/LConn3 -- T_171573029__Biloela_Substation/LConn3 -- bus223/LConn1
  G_119996556_Callide_Power_Station_A/RConn1 -- _CN_171573029_132000_CN_119996556_132000/RConn1
  G_119996556_Callide_Power_Station_A/RConn2 -- _CN_171573029_132000_CN_119996556_132000/RConn2
  _CN_171573029_132000_CN_119996556_132000/RConn3 -- G_119996556_Callide_Power_Station_A/RConn3 -- bus224/LConn1
  T_175020086__QR_Clayton_substation/LConn1 -- _CN_175017770_132000_CN_175020086_132000/RConn1
  T_175020086__QR_Clayton_substation/LConn2 -- _CN_175017770_132000_CN_175020086_132000/RConn2
  _CN_175017770_132000_CN_175020086_132000/RConn3 -- T_175020086__QR_Clayton_substation/LConn3 -- bus225/LConn1
  T_165709781__/LConn1 -- _CN_161829167_132000_CN_165709781_132000/RConn1
  T_165709781__/LConn2 -- _CN_161829167_132000_CN_165709781_132000/RConn2
  _CN_161829167_132000_CN_165709781_132000/RConn3 -- T_165709781__/LConn3 -- bus226/LConn1
  T_377141169__Charmhaven_Zone_Substation/LConn1 -- _CN_377141169_132000_CN_24024039_132000/LConn1
  T_377141169__Charmhaven_Zone_Substation/LConn2 -- _CN_377141169_132000_CN_24024039_132000/LConn2
  _CN_377141169_132000_CN_24024039_132000/LConn3 -- T_377141169__Charmhaven_Zone_Substation/LConn3 -- bus227/LConn1
  _CN_377141169_132000_CN_24024039_132000/RConn1 -- T_24024039__/RConn1 -- L_24024039/LConn1
  _CN_377141169_132000_CN_24024039_132000/RConn2 -- T_24024039__/RConn2 -- L_24024039/LConn2
  _CN_377141169_132000_CN_24024039_132000/RConn3 -- T_24024039__/RConn3 -- L_24024039/LConn3 -- bus228/LConn1
  T_218450415__/LConn1 -- _CN_175920440_132000_CN_218450415_132000/RConn1
  T_218450415__/LConn2 -- _CN_175920440_132000_CN_218450415_132000/RConn2
  _CN_175920440_132000_CN_218450415_132000/RConn3 -- T_218450415__/LConn3 -- bus229/LConn1
  _CN_54674751_132000_CN_432510474_132000/RConn1 -- T_432510474__Calliope_River_Substation/RConn1 -- L_432510474/LConn1
  _CN_54674751_132000_CN_432510474_132000/RConn2 -- T_432510474__Calliope_River_Substation/RConn2 -- L_432510474/LConn2
  _CN_54674751_132000_CN_432510474_132000/RConn3 -- T_432510474__Calliope_River_Substation/RConn3 -- L_432510474/LConn3 -- bus230/LConn1
  _CN_72231242_132000_CN_72231236_132000/RConn1 -- T_72231242__/LConn1 -- _CN_72231242_132000_CN_171581834_132000/LConn1 -- _CN_72231242_132000_CN_170840487_132000/RConn1
  _CN_72231242_132000_CN_72231236_132000/RConn2 -- T_72231242__/LConn2 -- _CN_72231242_132000_CN_171581834_132000/LConn2 -- _CN_72231242_132000_CN_170840487_132000/RConn2
  _CN_72231242_132000_CN_72231236_132000/RConn3 -- T_72231242__/LConn3 -- _CN_72231242_132000_CN_171581834_132000/LConn3 -- _CN_72231242_132000_CN_170840487_132000/RConn3 -- bus231/LConn1
  T_171581834__/LConn1 -- _CN_72231242_132000_CN_171581834_132000/RConn1
  T_171581834__/LConn2 -- _CN_72231242_132000_CN_171581834_132000/RConn2
  _CN_72231242_132000_CN_171581834_132000/RConn3 -- T_171581834__/LConn3 -- bus232/LConn1
  _CN_171846476_132000_CN_166113109_132000/LConn1 -- T_171846476__/LConn1 -- _CN_171846476_132000_CN_219209922_132000/LConn1
  _CN_171846476_132000_CN_166113109_132000/LConn2 -- T_171846476__/LConn2 -- _CN_171846476_132000_CN_219209922_132000/LConn2
  _CN_171846476_132000_CN_166113109_132000/LConn3 -- T_171846476__/LConn3 -- _CN_171846476_132000_CN_219209922_132000/LConn3 -- bus233/LConn1
  T_166113109__/LConn1 -- _CN_171846476_132000_CN_166113109_132000/RConn1
  T_166113109__/LConn2 -- _CN_171846476_132000_CN_166113109_132000/RConn2
  _CN_171846476_132000_CN_166113109_132000/RConn3 -- T_166113109__/LConn3 -- bus234/LConn1
  T_219209922__/LConn1 -- _CN_171846476_132000_CN_219209922_132000/RConn1
  T_219209922__/LConn2 -- _CN_171846476_132000_CN_219209922_132000/RConn2
  _CN_171846476_132000_CN_219209922_132000/RConn3 -- T_219209922__/LConn3 -- bus235/LConn1
  T_255775138_132000;33000_Outer_Harbour_Transmission_Substation/LConn1 -- _CN_142733661_132000_CN_255775138_132000/RConn1
  T_255775138_132000;33000_Outer_Harbour_Transmission_Substation/LConn2 -- _CN_142733661_132000_CN_255775138_132000/RConn2
  _CN_142733661_132000_CN_255775138_132000/RConn3 -- T_255775138_132000;33000_Outer_Harbour_Transmission_Substation/LConn3 -- bus236/LConn1
  T_46503657__Beechboro_Substation/LConn1 -- _CN_44187488_132000_CN_46503657_132000/RConn1
  T_46503657__Beechboro_Substation/LConn2 -- _CN_44187488_132000_CN_46503657_132000/RConn2
  _CN_44187488_132000_CN_46503657_132000/RConn3 -- T_46503657__Beechboro_Substation/LConn3 -- bus237/LConn1
  _CN_171189090_132000_CN_171980651_132000/LConn1 -- T_171189090_275000_275_kV_Ross/RConn1 -- L_171189090/LConn1
  _CN_171189090_132000_CN_171980651_132000/LConn2 -- T_171189090_275000_275_kV_Ross/RConn2 -- L_171189090/LConn2
  _CN_171189090_132000_CN_171980651_132000/LConn3 -- T_171189090_275000_275_kV_Ross/RConn3 -- L_171189090/LConn3 -- bus238/LConn1
  _CN_171189090_132000_CN_171980651_132000/RConn1 -- T_171980651__/LConn1 -- _CN_171189093_132000_CN_171980651_132000/LConn1
  _CN_171189090_132000_CN_171980651_132000/RConn2 -- T_171980651__/LConn2 -- _CN_171189093_132000_CN_171980651_132000/LConn2
  _CN_171189090_132000_CN_171980651_132000/RConn3 -- T_171980651__/LConn3 -- _CN_171189093_132000_CN_171980651_132000/LConn3 -- bus239/LConn1
  T_171189093__/LConn1 -- _CN_171189093_132000_CN_171980651_132000/RConn1
  T_171189093__/LConn2 -- _CN_171189093_132000_CN_171980651_132000/RConn2
  _CN_171189093_132000_CN_171980651_132000/RConn3 -- T_171189093__/LConn3 -- bus240/LConn1
  T_328487572__Birtinya_Substation/LConn1 -- _CN_328487572_132000_CN_328487570_132000/LConn1
  T_328487572__Birtinya_Substation/LConn2 -- _CN_328487572_132000_CN_328487570_132000/LConn2
  _CN_328487572_132000_CN_328487570_132000/LConn3 -- T_328487572__Birtinya_Substation/LConn3 -- bus241/LConn1
  T_328487570__Kawana_Substation/LConn1 -- _CN_328487572_132000_CN_328487570_132000/RConn1
  T_328487570__Kawana_Substation/LConn2 -- _CN_328487572_132000_CN_328487570_132000/RConn2
  _CN_328487572_132000_CN_328487570_132000/RConn3 -- T_328487570__Kawana_Substation/LConn3 -- bus242/LConn1
  T_373381185__Hume_Streets_Sub_Station/LConn1 -- _CN_373381185_132000_CN_171979185_132000/LConn1
  T_373381185__Hume_Streets_Sub_Station/LConn2 -- _CN_373381185_132000_CN_171979185_132000/LConn2
  _CN_373381185_132000_CN_171979185_132000/LConn3 -- T_373381185__Hume_Streets_Sub_Station/LConn3 -- bus243/LConn1
  _CN_373381185_132000_CN_171979185_132000/RConn1 -- T_171979185__/LConn1 -- _CN_171979185_132000_CN_259142988_132000/LConn1
  _CN_373381185_132000_CN_171979185_132000/RConn2 -- T_171979185__/LConn2 -- _CN_171979185_132000_CN_259142988_132000/LConn2
  _CN_373381185_132000_CN_171979185_132000/RConn3 -- T_171979185__/LConn3 -- _CN_171979185_132000_CN_259142988_132000/LConn3 -- bus244/LConn1
  T_284934380__/LConn1 -- _CN_284934380_132000_CN_175862605_132000/RConn1
  T_284934380__/LConn2 -- _CN_284934380_132000_CN_175862605_132000/RConn2
  _CN_284934380_132000_CN_175862605_132000/RConn3 -- T_284934380__/LConn3 -- bus245/LConn1
  T_259142988__/LConn1 -- _CN_171979185_132000_CN_259142988_132000/RConn1
  T_259142988__/LConn2 -- _CN_171979185_132000_CN_259142988_132000/RConn2
  _CN_171979185_132000_CN_259142988_132000/RConn3 -- T_259142988__/LConn3 -- bus246/LConn1
  T_229813242__/LConn1 -- _CN_166184400_132000_CN_229813242_132000/RConn1
  T_229813242__/LConn2 -- _CN_166184400_132000_CN_229813242_132000/RConn2
  _CN_166184400_132000_CN_229813242_132000/RConn3 -- T_229813242__/LConn3 -- bus247/LConn1
  T_229813239__/LConn1 -- _CN_166184400_132000_CN_229813239_132000/RConn1
  T_229813239__/LConn2 -- _CN_166184400_132000_CN_229813239_132000/RConn2
  _CN_166184400_132000_CN_229813239_132000/RConn3 -- T_229813239__/LConn3 -- bus248/LConn1
  _CN_223943114_220000_CN_223942734_220000/LConn1 -- T_223943114__/RConn1 -- L_223943114/LConn1
  _CN_223943114_220000_CN_223942734_220000/LConn2 -- T_223943114__/RConn2 -- L_223943114/LConn2
  _CN_223943114_220000_CN_223942734_220000/LConn3 -- T_223943114__/RConn3 -- L_223943114/LConn3 -- bus249/LConn1
  _CN_223943114_220000_CN_223942734_220000/RConn1 -- T_223942734__/LConn1 -- _CN_223942734_220000_CN_223940475_220000/LConn1
  _CN_223943114_220000_CN_223942734_220000/RConn2 -- T_223942734__/LConn2 -- _CN_223942734_220000_CN_223940475_220000/LConn2
  _CN_223943114_220000_CN_223942734_220000/RConn3 -- T_223942734__/LConn3 -- _CN_223942734_220000_CN_223940475_220000/LConn3 -- bus250/LConn1
  T_346232962__TOA_Elaine_Terminal_Station/LConn1 -- _CN_346232962_220000_CN_89180086_220000/LConn1
  T_346232962__TOA_Elaine_Terminal_Station/LConn2 -- _CN_346232962_220000_CN_89180086_220000/LConn2
  _CN_346232962_220000_CN_89180086_220000/LConn3 -- T_346232962__TOA_Elaine_Terminal_Station/LConn3 -- bus251/LConn1
  _CN_346232962_220000_CN_89180086_220000/RConn1 -- T_89180086__AusNet_Ballarat_Terminal_Station/LConn1 -- _CN_193910534_220000_CN_89180086_220000/LConn1 -- _CN_156598151_220000_CN_89180086_220000/LConn1
  _CN_346232962_220000_CN_89180086_220000/RConn2 -- T_89180086__AusNet_Ballarat_Terminal_Station/LConn2 -- _CN_193910534_220000_CN_89180086_220000/LConn2 -- _CN_156598151_220000_CN_89180086_220000/LConn2
  _CN_346232962_220000_CN_89180086_220000/RConn3 -- T_89180086__AusNet_Ballarat_Terminal_Station/LConn3 -- _CN_193910534_220000_CN_89180086_220000/LConn3 -- _CN_156598151_220000_CN_89180086_220000/LConn3 -- bus252/LConn1
  _CN_88187651_220000_CN_104719368_220000/LConn1 -- T_88187651__Hadspen_Substation/LConn1 -- _CN_88187651_220000_CN_174441055_220000/LConn1
  _CN_88187651_220000_CN_104719368_220000/LConn2 -- T_88187651__Hadspen_Substation/LConn2 -- _CN_88187651_220000_CN_174441055_220000/LConn2
  _CN_88187651_220000_CN_104719368_220000/LConn3 -- T_88187651__Hadspen_Substation/LConn3 -- _CN_88187651_220000_CN_174441055_220000/LConn3 -- bus253/LConn1
  _CN_88187651_220000_CN_104719368_220000/RConn1 -- T_104719368__George_Town_Substation/LConn1 -- Basslink_CN_104719368_220000_CN_104720150_220000/LConn1
  _CN_88187651_220000_CN_104719368_220000/RConn2 -- T_104719368__George_Town_Substation/LConn2 -- Basslink_CN_104719368_220000_CN_104720150_220000/LConn2
  _CN_88187651_220000_CN_104719368_220000/RConn3 -- T_104719368__George_Town_Substation/LConn3 -- Basslink_CN_104719368_220000_CN_104720150_220000/LConn3 -- bus254/LConn1
  _CN_88187651_220000_CN_174441055_220000/RConn1 -- T_174441055__/LConn1 -- _CN_88191017_220000_CN_174441055_220000/LConn1
  _CN_88187651_220000_CN_174441055_220000/RConn2 -- T_174441055__/LConn2 -- _CN_88191017_220000_CN_174441055_220000/LConn2
  _CN_88187651_220000_CN_174441055_220000/RConn3 -- T_174441055__/LConn3 -- _CN_88191017_220000_CN_174441055_220000/LConn3 -- bus255/LConn1
  _CN_107265156_220000_CN_286063160_220000/LConn1 -- T_107265156__/LConn1 -- _CN_107265156_220000_CN_107270533_220000/LConn1 -- _CN_107265156_220000_CN_239029214_220000/LConn1 -- _CN_107265156_220000_CN_172236849_220000/LConn1 -- _CN_107265156_220000_CN_56234037_220000/LConn1
  _CN_107265156_220000_CN_286063160_220000/LConn2 -- T_107265156__/LConn2 -- _CN_107265156_220000_CN_107270533_220000/LConn2 -- _CN_107265156_220000_CN_239029214_220000/LConn2 -- _CN_107265156_220000_CN_172236849_220000/LConn2 -- _CN_107265156_220000_CN_56234037_220000/LConn2
  _CN_107265156_220000_CN_286063160_220000/LConn3 -- T_107265156__/LConn3 -- _CN_107265156_220000_CN_107270533_220000/LConn3 -- _CN_107265156_220000_CN_239029214_220000/LConn3 -- _CN_107265156_220000_CN_172236849_220000/LConn3 -- bus256/LConn1 -- _CN_107265156_220000_CN_56234037_220000/LConn3
  _CN_107265156_220000_CN_286063160_220000/RConn1 -- T_286063160__/RConn1 -- _CN_286063160_220000_CN_205163985_220000/LConn1 -- L_286063160/LConn1
  _CN_107265156_220000_CN_286063160_220000/RConn2 -- T_286063160__/RConn2 -- _CN_286063160_220000_CN_205163985_220000/LConn2 -- L_286063160/LConn2
  _CN_107265156_220000_CN_286063160_220000/RConn3 -- T_286063160__/RConn3 -- _CN_286063160_220000_CN_205163985_220000/LConn3 -- L_286063160/LConn3 -- bus257/LConn1
  _CN_107265156_220000_CN_56234037_220000/RConn1 -- T_56234037__Eildon_Terminal_Station/LConn1 -- _CN_56234037_220000_CN_64943050_220000/LConn1
  _CN_107265156_220000_CN_56234037_220000/RConn2 -- T_56234037__Eildon_Terminal_Station/LConn2 -- _CN_56234037_220000_CN_64943050_220000/LConn2
  _CN_107265156_220000_CN_56234037_220000/RConn3 -- T_56234037__Eildon_Terminal_Station/LConn3 -- _CN_56234037_220000_CN_64943050_220000/LConn3 -- bus258/LConn1
  G_107270533_West_Kiewa_Power_Station/RConn1 -- _CN_107265156_220000_CN_107270533_220000/RConn1
  G_107270533_West_Kiewa_Power_Station/RConn2 -- _CN_107265156_220000_CN_107270533_220000/RConn2
  _CN_107265156_220000_CN_107270533_220000/RConn3 -- G_107270533_West_Kiewa_Power_Station/RConn3 -- bus259/LConn1
  G_239029214_Dartmouth_Power_Station/RConn1 -- _CN_107265156_220000_CN_239029214_220000/RConn1
  G_239029214_Dartmouth_Power_Station/RConn2 -- _CN_107265156_220000_CN_239029214_220000/RConn2
  _CN_107265156_220000_CN_239029214_220000/RConn3 -- G_239029214_Dartmouth_Power_Station/RConn3 -- bus260/LConn1
  G_172236849_/RConn1 -- _CN_107265156_220000_CN_172236849_220000/RConn1
  G_172236849_/RConn2 -- _CN_107265156_220000_CN_172236849_220000/RConn2
  _CN_107265156_220000_CN_172236849_220000/RConn3 -- G_172236849_/RConn3 -- bus261/LConn1
  T_193910534__/LConn1 -- _CN_193910534_220000_CN_89180086_220000/RConn1
  T_193910534__/LConn2 -- _CN_193910534_220000_CN_89180086_220000/RConn2
  _CN_193910534_220000_CN_89180086_220000/RConn3 -- T_193910534__/LConn3 -- bus262/LConn1
  _CN_156598151_220000_CN_49455810_220000/LConn1 -- T_156598151__AusNet_Terang_Terminal_Station/LConn1 -- _CN_156598151_220000_CN_89180086_220000/RConn1
  _CN_156598151_220000_CN_49455810_220000/LConn2 -- T_156598151__AusNet_Terang_Terminal_Station/LConn2 -- _CN_156598151_220000_CN_89180086_220000/RConn2
  _CN_156598151_220000_CN_49455810_220000/LConn3 -- T_156598151__AusNet_Terang_Terminal_Station/LConn3 -- _CN_156598151_220000_CN_89180086_220000/RConn3 -- bus263/LConn1
  _CN_156598151_220000_CN_49455810_220000/RConn1 -- T_49455810__Moorabool_Terminal_Station/RConn1 -- _CN_244141232_220000_CN_49455810_220000/LConn1 -- L_49455810/LConn1
  _CN_156598151_220000_CN_49455810_220000/RConn2 -- T_49455810__Moorabool_Terminal_Station/RConn2 -- _CN_244141232_220000_CN_49455810_220000/LConn2 -- L_49455810/LConn2
  _CN_156598151_220000_CN_49455810_220000/RConn3 -- T_49455810__Moorabool_Terminal_Station/RConn3 -- _CN_244141232_220000_CN_49455810_220000/LConn3 -- L_49455810/LConn3 -- bus264/LConn1
  T_104720150__Basslink_DC_AC_convertor_station/LConn1 -- Basslink_CN_104719368_220000_CN_104720150_220000/RConn1
  T_104720150__Basslink_DC_AC_convertor_station/LConn2 -- Basslink_CN_104719368_220000_CN_104720150_220000/RConn2
  Basslink_CN_104719368_220000_CN_104720150_220000/RConn3 -- T_104720150__Basslink_DC_AC_convertor_station/LConn3 -- bus265/LConn1
